simulink model "V1"  (R2025b)
settings: Solver=VariableStepAuto  StartTime=0.0  StopTime=3600*9  RelTol=1e-3
model workspace (MAT data in the model file):
  COP = 3.9
  Delayfan = [30 1]
  P1 = 1.05
  P2 = 1.91
  P3 = 1.91
  P4 = 1.05
  Q_Cond = 4.361
  Q_Evap = 3.471
  T1 = 12
  T2 = 37.72
  T3 = 29.61
  T4 = 7.9
  T_Enviroment_C = 27.5
  T_Room_int_C = 28.6
  T_Tank_int_c = 30
  Wall_h_in = 12
  Wall_h_out = 38
  h1 = 522.3
  h2 = 528.6
  h3 = 253.4
  h4 = 253.4
  m_dot = 0.014
libraries: fl_lib x102, nesl_utility x62, SimscapeFluids_lib x31
(part 1 of 4)
settings Model: Creator=acer  LastModifiedBy=acer

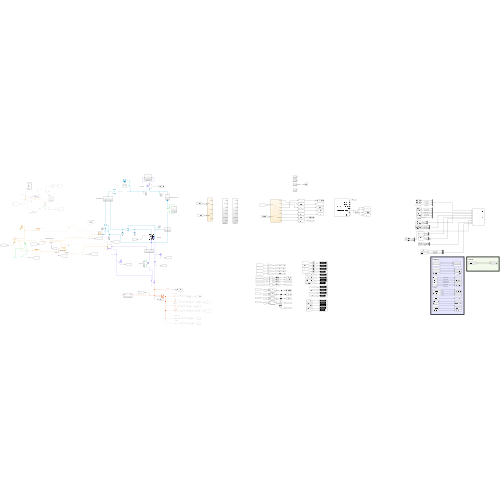
[thumbnail: Simulink's stored preview of the top-level diagram]
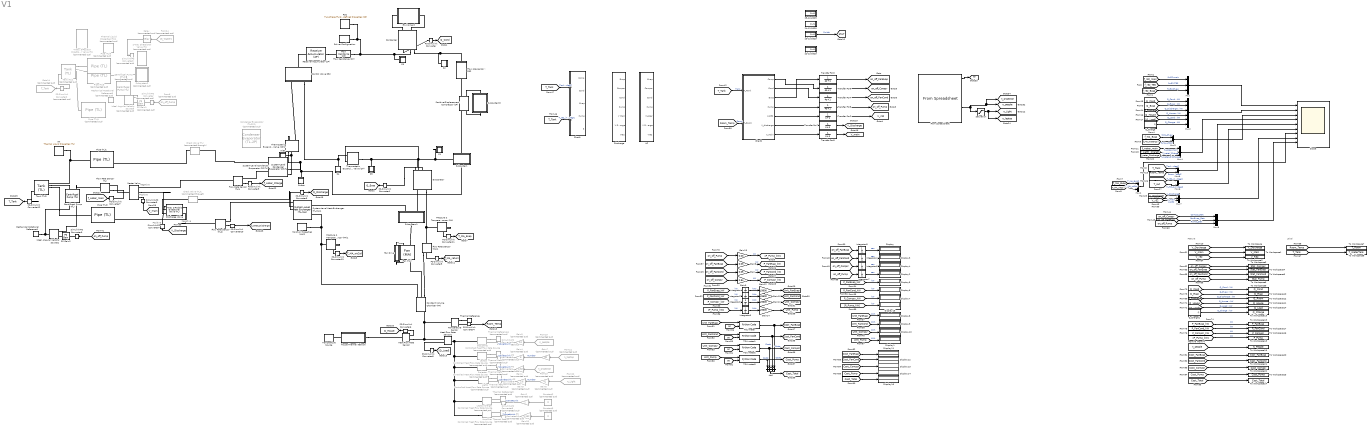
== system V1 ==
  note: Feature
  note: Positive
  note: Negative
  note: Positive
  note: Negative
  note: Label
  2-Way Directional Valve (TL) : SimscapeFluids_lib/Thermal Liquid/Valves & Orifices/Directional Control Valves/2-Way Directional Valve (TL)  Commented=on  valve_spec=fluids.thermal_liquid.valves.directional_control_valves.enum.ValveSpec.Linear  S_max=0.01 m  del_S_max=0.01 m  area_max=0.015 m^2  area_leak=1e-6 m^2  del_S_TLU=[0, .002, .004, .007, .017] m  valve_area_TLU=[1e-09, 2.0352e-07, 4.0736e-05, .00011438, .00034356] m^2  del_S_flow_TLU=[0, .002, .004, .007, .017] m  p_diff_TLU=[.3, .5, .7] MPa  vol_flow_TLU=1e-3 * [1.7e-05, 2e-05, 2.6e-05; .0035, .0045, .0053; .7, .9, 1.06; 1.96, 2.5, 3; 6, 7.7, 9.13] m^3/s  mdot_TLU=[1.7e-05, 2e-05, 2.6e-05; .0035, .0045, .0053; .7, .9, 1.06; 1.96, 2.5, 3; 6, 7.7, 9.13] kg/s  T_ref_in=293.15 K  p_ref_in=0.101325 MPa  Cd=0.9  Re_c=150  smoothing_factor=0.01  pressure_recovery=false  area=0.016 m^2
      settings: InternalSimscapePortConfiguration="{\"Bottom\":[],\"Left\":[{\"id\":\"A\",\"label\":\"A\",\"type\":\"foundation.thermal_liquid.thermal_liquid\"}],\"Right\":[{\"id\":\"S\",\"label\":\"S\",\"type\":\"input\"},{\"id\":\"B\",\"label\":\"B\",\"type\":\"foundation.thermal_liquid.thermal_liquid\"}],\"Top\":[]}"
  22-12-2025 : Subsystem
  23-12-2025 : Subsystem
  24-12-2025 : Subsystem
  25-12-2025 : Subsystem
  4-Way 3-Position Directional Valve (TL) : SimscapeFluids_lib/Thermal Liquid/Valves & Orifices/Directional Control Valves/4-Way 3-Position Directional Valve (TL)  Commented=on  open_orifices_pos=fluids.thermal_liquid.valves.directional_control_valves.enum.OpenOrifices4WayPosNeg.PA  open_orifices_neu=fluids.thermal_liquid.valves.directional_control_valves.enum.OpenOrifices4WayNeu.AT_BT  open_orifices_neg=fluids.thermal_liquid.valves.directional_control_valves.enum.OpenOrifices4WayPosNeg.PA_BT  neutral_assert_action=simscape.enum.assert.action.warn  area_spec=fluids.thermal_liquid.valves.directional_control_valves.enum.area_spec.identical  valve_spec=fluids.thermal_liquid.valves.directional_control_valves.enum.ValveSpec.Linear  del_S_max=0.005 m  area_max=1e-4 m^2  del_S_TLU=[0, .00125, .0025, .00375, .005] m  valve_area_TLU=[1e-10, 1e-05, 4e-05, 6e-05, .0001] m^2  del_S_flow_TLU=[0, .00125, .0025, .00375, .005] m  p_diff_TLU=[-.1, .3, .5, .7] MPa  vol_flow_TLU=[-1e-08, 2.2e-08, 2.8e-08, 3.4e-08; -9e-06, .00015, .0002, .00024; -.00036, .00063, .00081, .00096; -.00054, .00094, .0012, .0014; -.00091, .0016, .002, .0024] m^3/s  mdot_TLU=[-1e-05, 1.7e-05, 2e-05, 2.6e-05; -.009, .0035, .0045, .0053; -.36, .7, .9, 1.06; -.54, 1.96, 2.5, 3; -.91, 6, 7.7, 9.13] kg/s  p_diff_TLU_const=[-.1, .3, .5, .7] MPa  vol_flow_TLU_const=[-.0009, .0016, .002, .0024] m^3/s  mdot_TLU_const=[-.9, 1.6, 2, 2.4] kg/s  area_const=1e-4 m^2  T_ref_in=293.15 K  p_ref_in=0.101325 MPa  area_leak=1e-10 m^2  area=0.01 m^2  Cd=0.64  Re_c=150  smoothing_factor=0.01  pressure_recovery=false  S_max_PA=7.5e-3 m  del_S_max_PA=0.005 m  area_max_PA=1e-4 m^2  del_S_TLU_PA=[0, .00125, .0025, .00375, .005] m  valve_area_TLU_PA=[1e-10, 1e-05, 4e-05, 6e-05, .0001] m^2  del_S_flow_TLU_PA=[0, .00125, .0025, .00375, .005] m  p_diff_TLU_PA=[-.1, .3, .5, .7] MPa  vol_flow_TLU_PA=[-1e-08, 2.2e-08, 2.8e-08, 3.4e-08; -9e-06, .00015, .0002, .00024; -.00036, .00063, .00081, .00096; -.00054, .00094, .0012, .0014; -.00091, .0016, .002, .0024] m^3/s  mdot_TLU_PA=[-1e-05, 1.7e-05, 2e-05, 2.6e-05; -.009, .0035, .0045, .0053; -.36, .7, .9, 1.06; -.54, 1.96, 2.5, 3; -.91, 6, 7.7, 9.13] kg/s  area_const_PA=1e-4 m^2  p_diff_TLU_const_PA=[-.1, .3, .5, .7] MPa  vol_flow_TLU_const_PA=[-.0009, .0016, .002, .0024] m^3/s  mdot_TLU_const_PA=[-.9, 1.6, 2, 2.4] kg/s  S_max_PB=-7.5e-3 m  del_S_max_PB=0.005 m  area_max_PB=1e-4 m^2  del_S_TLU_PB=[0, .00125, .0025, .00375, .005] m  valve_area_TLU_PB=[1e-10, 1e-05, 4e-05, 6e-05, .0001] m^2  del_S_flow_TLU_PB=[0, .00125, .0025, .00375, .005] m  p_diff_TLU_PB=[-.1, .3, .5, .7] MPa  vol_flow_TLU_PB=[-1e-08, 2.2e-08, 2.8e-08, 3.4e-08; -9e-06, .00015, .0002, .00024; -.00036, .00063, .00081, .00096; -.00054, .00094, .0012, .0014; -.00091, .0016, .002, .0024] m^3/s  mdot_TLU_PB=[-1e-05, 1.7e-05, 2e-05, 2.6e-05; -.009, .0035, .0045, .0053; -.36, .7, .9, 1.06; -.54, 1.96, 2.5, 3; -.91, 6, 7.7, 9.13] kg/s  area_const_PB=1e-4 m^2  p_diff_TLU_const_PB=[-.1, .3, .5, .7] MPa  vol_flow_TLU_const_PB=[-.0009, .0016, .002, .0024] m^3/s  mdot_TLU_const_PB=[-.9, 1.6, 2, 2.4] kg/s  S_max_AB=7.5e-3 m  del_S_max_AB=0.005 m  area_max_AB=1e-4 m^2  del_S_TLU_AB=[0, .00125, .0025, .00375, .005] m  valve_area_TLU_AB=[1e-10, 1e-05, 4e-05, 6e-05, .0001] m^2  del_S_flow_TLU_AB=[0, .00125, .0025, .00375, .005] m  p_diff_TLU_AB=[-.1, .3, .5, .7] MPa  vol_flow_TLU_AB=[-1e-08, 2.2e-08, 2.8e-08, 3.4e-08; -9e-06, .00015, .0002, .00024; -.00036, .00063, .00081, .00096; -.00054, .00094, .0012, .0014; -.00091, .0016, .002, .0024] m^3/s  mdot_TLU_AB=[-1e-05, 1.7e-05, 2e-05, 2.6e-05; -.009, .0035, .0045, .0053; -.36, .7, .9, 1.06; -.54, 1.96, 2.5, 3; -.91, 6, 7.7, 9.13] kg/s  area_const_AB=1e-4 m^2  p_diff_TLU_const_AB=[-.1, .3, .5, .7] MPa  vol_flow_TLU_const_AB=[-.0009, .0016, .002, .0024] m^3/s  mdot_TLU_const_AB=[-.9, 1.6, 2, 2.4] kg/s  S_max_AT=-7.5e-3 m  del_S_max_AT=0.005 m  area_max_AT=1e-4 m^2  del_S_TLU_AT=[0, .00125, .0025, .00375, .005] m  valve_area_TLU_AT=[1e-10, 1e-05, 4e-05, 6e-05, .0001] m^2  del_S_flow_TLU_AT=[0, .00125, .0025, .00375, .005] m  p_diff_TLU_AT=[-.1, .3, .5, .7] MPa  vol_flow_TLU_AT=[-1e-08, 2.2e-08, 2.8e-08, 3.4e-08; -9e-06, .00015, .0002, .00024; -.00036, .00063, .00081, .00096; -.00054, .00094, .0012, .0014; -.00091, .0016, .002, .0024] m^3/s  mdot_TLU_AT=[-1e-05, 1.7e-05, 2e-05, 2.6e-05; -.009, .0035, .0045, .0053; -.36, .7, .9, 1.06; -.54, 1.96, 2.5, 3; -.91, 6, 7.7, 9.13] kg/s  area_const_AT=1e-4 m^2  p_diff_TLU_const_AT=[-.1, .3, .5, .7] MPa  vol_flow_TLU_const_AT=[-.0009, .0016, .002, .0024] m^3/s  mdot_TLU_const_AT=[-.9, 1.6, 2, 2.4] kg/s  S_max_BT=7.5e-3 m  del_S_max_BT=0.005 m  area_max_BT=1e-4 m^2  del_S_TLU_BT=[0, .00125, .0025, .00375, .005] m  valve_area_TLU_BT=[1e-10, 1e-05, 4e-05, 6e-05, .0001] m^2  del_S_flow_TLU_BT=[0, .00125, .0025, .00375, .005] m  p_diff_TLU_BT=[-.1, .3, .5, .7] MPa  vol_flow_TLU_BT=[-1e-08, 2.2e-08, 2.8e-08, 3.4e-08; -9e-06, .00015, .0002, .00024; -.00036, .00063, .00081, .00096; -.00054, .00094, .0012, .0014; -.00091, .0016, .002, .0024] m^3/s  mdot_TLU_BT=[-1e-05, 1.7e-05, 2e-05, 2.6e-05; -.009, .0035, .0045, .0053; -.36, .7, .9, 1.06; -.54, 1.96, 2.5, 3; -.91, 6, 7.7, 9.13] kg/s  area_const_BT=1e-4 m^2  p_diff_TLU_const_BT=[-.1, .3, .5, .7] MPa  vol_flow_TLU_const_BT=[-.0009, .0016, .002, .0024] m^3/s  mdot_TLU_const_BT=[-.9, 1.6, 2, 2.4] kg/s  S_max_PT=0 m  del_S_max_PT=0.005 m  area_max_PT=1e-4 m^2  del_S_TLU_PT=[0, .00125, .0025, .00375, .005] m  valve_area_TLU_PT=[1e-10, 1e-05, 4e-05, 6e-05, .0001] m^2  del_S_flow_TLU_PT=[0, .00125, .0025, .00375, .005] m  p_diff_TLU_PT=[-.1, .3, .5, .7] MPa  vol_flow_TLU_PT=[-1e-08, 2.2e-08, 2.8e-08, 3.4e-08; -9e-06, .00015, .0002, .00024; -.00036, .00063, .00081, .00096; -.00054, .00094, .0012, .0014; -.00091, .0016, .002, .0024] m^3/s  mdot_TLU_PT=[-1e-05, 1.7e-05, 2e-05, 2.6e-05; -.009, .0035, .0045, .0053; -.36, .7, .9, 1.06; -.54, 1.96, 2.5, 3; -.91, 6, 7.7, 9.13] kg/s
      settings: InternalSimscapePortConfiguration="{\"Bottom\":[],\"Left\":[{\"id\":\"A\",\"label\":\"A\",\"type\":\"foundation.thermal_liquid.thermal_liquid\"},{\"id\":\"B\",\"label\":\"B\",\"type\":\"foundation.thermal_liquid.thermal_liquid\"}],\"Right\":[{\"id\":\"S\",\"label\":\"S\",\"type\":\"input\"},{\"id\":\"P\",\"label\":\"P\",\"type\":\"foundation.thermal_liquid.thermal_liquid\"},{\"id\":\"T\",\"label\":\"T\",\"type\":\"foundation.thermal_liquid.thermal_liquid\"}],\"Top\":[]}"
  AC : Subsystem
  Add : Sum  Inputs=++++
  Amplifier : fl_lib/Thermal/Thermal Sources/Controlled Heat Flow Rate Source  Commented=on
  Centrifugal Pump (TL) : SimscapeFluids_lib/Thermal Liquid/Pumps & Motors/Centrifugal Pump (TL)  pump_parameterization=fluids.thermal_liquid.pumps_motors.enum.CentrifugalPumpParameterization.Nominal  capacity_ref_nominal=45 lpm  head_ref_nominal=40 m  power_ref_nominal=0.85 kW  head_ref_max=60 m  capacity_ref_max=80 lpm  omega_ref_analytic=1770 rpm  flow_rate_1D_TLU=[16.67, 30, 40, 53.33, 66.67, 83.33] lpm  head_1D_TLU=[50, 47.5, 45, 40, 35, 25] m  power_1D_TLU=[.6, .75, .85, .93, .98, .99] kW  omega_ref_1D=3500 rpm  rho_ref_1D=998.21 kg/m^3  omega_threshold_factor=1e-2  flow_rate_2D_TLU=[16.67, 23.33, 30, 40, 53.33, 60] lpm  omega_2D_TLU=[2450, 2800, 3150, 3500] rpm  head_2D_TLU=[25, 32.7, 42.5, 50; 24, 31.7, 41, 49; 22.7, 30.5, 39, 47.5; 20, 28, 36, 45; 15.7, 24, 32, 40; 12.5, 21, 29.5, 37.5] m  power_2D_TLU=[.28, .38, .5, .6; .31, .41, .55, .68; .33, .44, .6, .75; .36, .48, .65, .83; .38, .53, .72, .93; .39, .55, .75, .97] kW  rho_ref_2D=998.21 kg/m^3  diameter_ratio=1  mech_orientation=fluids.thermal_liquid.pumps_motors.enum.CentrifugalPumpMechOrientation.Positive  area=0.01 m^2  operation_check=simscape.enum.assert.action.none
      settings: InternalSimscapePortConfiguration="{\"Bottom\":[],\"Left\":[{\"id\":\"A\",\"label\":\"A\",\"type\":\"foundation.thermal_liquid.thermal_liquid\"},{\"id\":\"B\",\"label\":\"B\",\"type\":\"foundation.thermal_liquid.thermal_liquid\"}],\"Right\":[{\"id\":\"R\",\"label\":\"R\",\"type\":\"foundation.mechanical.rotational.rotational\"},{\"id\":\"C\",\"label\":\"C\",\"type\":\"foundation.mechanical.rotational.rotational\"}],\"Top\":[]}"
  Centrifugal Pump (TL)2 : SimscapeFluids_lib/Thermal Liquid/Pumps & Motors/Centrifugal Pump (TL)  Commented=on  pump_parameterization=fluids.thermal_liquid.pumps_motors.enum.CentrifugalPumpParameterization.Nominal  capacity_ref_nominal=10 lpm  head_ref_nominal=5 m  power_ref_nominal=0.01 kW  head_ref_max=9 m  capacity_ref_max=11 lpm  omega_ref_analytic=1500 rpm  flow_rate_1D_TLU=[16.67, 30, 40, 53.33, 66.67, 83.33] lpm  head_1D_TLU=[50, 47.5, 45, 40, 35, 25] m  power_1D_TLU=[.6, .75, .85, .93, .98, .99] kW  omega_ref_1D=3500 rpm  rho_ref_1D=998.21 kg/m^3  omega_threshold_factor=1e-2  flow_rate_2D_TLU=[16.67, 23.33, 30, 40, 53.33, 60] lpm  omega_2D_TLU=[2450, 2800, 3150, 3500] rpm  head_2D_TLU=[25, 32.7, 42.5, 50; 24, 31.7, 41, 49; 22.7, 30.5, 39, 47.5; 20, 28, 36, 45; 15.7, 24, 32, 40; 12.5, 21, 29.5, 37.5] m  power_2D_TLU=[.28, .38, .5, .6; .31, .41, .55, .68; .33, .44, .6, .75; .36, .48, .65, .83; .38, .53, .72, .93; .39, .55, .75, .97] kW  rho_ref_2D=998.21 kg/m^3  diameter_ratio=1  mech_orientation=fluids.thermal_liquid.pumps_motors.enum.CentrifugalPumpMechOrientation.Positive  area=7.8e-5 m^2  operation_check=simscape.enum.assert.action.none
      settings: InternalSimscapePortConfiguration="{\"Bottom\":[],\"Left\":[{\"id\":\"A\",\"label\":\"A\",\"type\":\"foundation.thermal_liquid.thermal_liquid\"},{\"id\":\"B\",\"label\":\"B\",\"type\":\"foundation.thermal_liquid.thermal_liquid\"}],\"Right\":[{\"id\":\"R\",\"label\":\"R\",\"type\":\"foundation.mechanical.rotational.rotational\"},{\"id\":\"C\",\"label\":\"C\",\"type\":\"foundation.mechanical.rotational.rotational\"}],\"Top\":[]}"
  Chart1 : Stateflow chart  TreatAsAtomicUnit=on
  Chart2 : Stateflow chart  TreatAsAtomicUnit=on
  Check Valve (TL) : SimscapeFluids_lib/Thermal Liquid/Valves & Orifices/Directional Control Valves/Check Valve (TL)  Commented=through  opening_spec=fluids.thermal_liquid.valves.enum.PressureOpeningSpec.Linear  pressure_spec=fluids.thermal_liquid.valves.enum.PressureControlSpec.PressureDifferential  p_crack_gauge=0.1 MPa  p_crack_differential=0.01 MPa  press_max_gauge=0.2 MPa  press_max_differential=0.02 MPa  area_max=1e-4 m^2  area_leak=1e-10 m^2  p_diff_TLU=[0.01 : 0.01 : 0.1] MPa  valve_area_TLU=[1e-10, 1e-05, 2e-05, 3e-05, 4e-05, 5e-05, 6e-05, 7.5e-05, 8.5e-05, .0001] m^2  vol_flow_TLU=[.000358, .045, .11, .191, .284, .39, .505, .63, .764, .905] .* 1e-3 m^3/s  area=0.01 m^2  Cd=0.64  Re_c=150  smoothing_factor=0.01  pressure_recovery=false  opening_dynamics=false  tau=0.1 s
      settings: InternalSimscapePortConfiguration="{\"Bottom\":[],\"Left\":[{\"id\":\"A\",\"label\":\"A\",\"type\":\"foundation.thermal_liquid.thermal_liquid\"}],\"Right\":[{\"id\":\"B\",\"label\":\"B\",\"type\":\"foundation.thermal_liquid.thermal_liquid\"}],\"Top\":[]}"
  Check Valve (TL)1 : SimscapeFluids_lib/Thermal Liquid/Valves & Orifices/Directional Control Valves/Check Valve (TL)  Commented=through  opening_spec=fluids.thermal_liquid.valves.enum.PressureOpeningSpec.Linear  pressure_spec=fluids.thermal_liquid.valves.enum.PressureControlSpec.PressureDifferential  p_crack_gauge=0.1 MPa  p_crack_differential=0.01 MPa  press_max_gauge=0.2 MPa  press_max_differential=0.02 MPa  area_max=1e-4 m^2  area_leak=1e-10 m^2  p_diff_TLU=[0.01 : 0.01 : 0.1] MPa  valve_area_TLU=[1e-10, 1e-05, 2e-05, 3e-05, 4e-05, 5e-05, 6e-05, 7.5e-05, 8.5e-05, .0001] m^2  vol_flow_TLU=[.000358, .045, .11, .191, .284, .39, .505, .63, .764, .905] .* 1e-3 m^3/s  area=0.01 m^2  Cd=0.64  Re_c=150  smoothing_factor=0.01  pressure_recovery=false  opening_dynamics=false  tau=0.1 s
      settings: InternalSimscapePortConfiguration="{\"Bottom\":[],\"Left\":[{\"id\":\"A\",\"label\":\"A\",\"type\":\"foundation.thermal_liquid.thermal_liquid\"}],\"Right\":[{\"id\":\"B\",\"label\":\"B\",\"type\":\"foundation.thermal_liquid.thermal_liquid\"}],\"Top\":[]}"
  Condenser : SimscapeFluids_lib/Heat Exchangers/Two-Phase Fluid - Moist Air/System-Level Condenser Evaporator (2P-MA)  flow_arrangement=fluids.heat_exchangers.enum.SystemLevelFlowArrangement2PMA.Counter  wall_thermal_mass=false  mass_wall=1 kg  cp_wall=490 J/(K*kg)  nominal_init_wall=true  T_wall_init=293.15 K  area_A1=0.01 m^2  area_B1=0.01 m^2  area_A2=0.01 m^2  area_B2=0.01 m^2  operating_condition_2P=fluids.heat_exchangers.enum.SystemLevelOperatingCondition2PMA.Condenser  mdot_nominal_2P=m_dot kg/s  delta_p_nominal_2P=0.045 MPa  pressure_spec_cond_2P=fluids.heat_exchangers.enum.SystemLevelPressureSpecCondenser2P.InletPressure  pressure_spec_evap_2P=fluids.heat_exchangers.enum.SystemLevelPressureSpecEvaporator2P.InletPressure  p_in_nominal_2P=P2 MPa  T_cond_nominal_2P=313.15 K  T_evap_nominal_2P=243.15 K  inlet_spec_2P=fluids.heat_exchangers.enum.SystemLevelInletSpec2P.Enthalpy  T_in_nominal_2P=333.15 K  h_in_nominal_2P=h2 kJ/kg  x_in_nominal_2P=1  capacity_spec_2P=fluids.heat_exchangers.enum.SystemLevelCapacitySpec.HeatTransfer  Q_nominal=m_dot*(h2-h3) kW  outlet_spec_cond_2P=fluids.heat_exchangers.enum.SystemLevelOutletSpecCondenser2P.Enthalpy  outlet_spec_evap_2P=fluids.heat_exchangers.enum.SystemLevelOutletSpecEvaporator2P.Enthalpy  delta_T_sub_nominal_2P=5 deltaK  delta_T_sup_nominal_2P=5 deltaK  h_out_nominal_2P=250 kJ/kg  x_out_nominal_2P=0  volume_2P=0.001 m^3  nominal_init_2P=true  energy_spec_2P=foundation.enum.energy_spec.enthalpy  p_init_2P=0.101325 MPa  T_init_2P=293.15 K  x_init_2P=0.5  alpha_init_2P=0.5  h_init_2P=1500 kJ/kg  u_init_2P=1500 kJ/kg  mdot_nominal_MA=5 kg/s  delta_p_nominal_MA=0.001 MPa  p_in_nominal_MA=0.101325 MPa  T_in_nominal_MA=T_Enviroment_C+273.15 K  inlet_humidity_spec_MA=foundation.enum.HumiditySpec.RelativeHumidity  RH_in_nominal_MA=0.5  x_w_in_nominal_MA=0.01  y_w_in_nominal_MA=0.01  HR_in_nominal_MA=0.01  Tw_in_nominal_MA=287 K  inlet_trace_gas_spec_MA=foundation.enum.trace_gas_spec.mass_fraction  x_g_in_nominal_MA=0.001  y_g_in_nominal_MA=0.001  volume_MA=0.1 m^3  nominal_init_MA=true  p_init_MA=0.101325 MPa  T_init_MA=293.15 K  humidity_spec_MA=foundation.enum.HumiditySpec.RelativeHumidity  RH_init_MA=0.5  x_w_init_MA=0.01  y_w_init_MA=0.01  HR_init_MA=0.01  Tw_init_MA=287 K  trace_gas_spec_MA=foundation.enum.trace_gas_spec.mass_fraction  x_g_init_MA=0.001  y_g_init_MA=0.001  r_d_init_MA=0  RH_ws_MA=1  time_constant_cond_MA=1e-3 s  time_constant_evap_MA=1e-3 s  fraction_entrained_MA=1  a_liq_2P=0.023  a_mix_2P=0.005  a_vap_2P=0.023  b_2P=0.8  c_2P=0.33  a_MA=0.023  b_MA=0.8  c_MA=0.33
      settings: InternalSimscapePortConfiguration="{\"Bottom\":[],\"Left\":[{\"id\":\"A1\",\"label\":\"A1\",\"type\":\"foundation.two_phase_fluid.two_phase_fluid\"},{\"id\":\"B1\",\"label\":\"B1\",\"type\":\"foundation.two_phase_fluid.two_phase_fluid\"}],\"Right\":[{\"id\":\"A2\",\"label\":\"A2\",\"type\":\"foundation.moist_air.moist_air\"},{\"id\":\"B2\",\"label\":\"B2\",\"type\":\"foundation.moist_air.moist_air\"}],\"Top\":[{\"id\":\"Q1\",\"label\":\"Q1\",\"type\":\"output\"},{\"id\":\"Q2\",\"label\":\"Q2\",\"type\":\"output\"},{\"id\":\"W\",\"label\":\"W\",\"type\":\"output\"}]}"
  Condenser Evaporator (TL-2P)1 : SimscapeFluids_lib/Heat Exchangers/Two-Phase Fluid - Thermal Liquid/Condenser Evaporator (TL-2P)  Commented=on  flow_arrangement=fluids.heat_exchangers.enum.FlowArrangementTL2P.Counter  cross_flow_arrangement=fluids.heat_exchangers.enum.CrossFlowArrangementTL2P.UnmixedUnmixed  R_wall=0.1 K/kW  wall_thermal_mass=true  mass_wall=4 kg  cp_wall=600 J/(K*kg)  area_A1=0.01 m^2  area_B1=0.01 m^2  area_A2=0.01 m^2  area_B2=0.01 m^2  flow_geometry_TL=fluids.heat_exchangers.enum.FlowGeometryTL.InsideTubes  tube_num_TL=30  tube_length_TL=2 m  tube_cross_section_TL=fluids.heat_exchangers.enum.TubeCrossSection.Circular  tube_diameter_TL=0.01 m  tube_width_TL=0.05 m  tube_height_TL=0.05 m  tube_inner_diameter_TL=0.05 m  tube_outer_diameter_TL=0.1 m  tube_flow_area_TL=0.002 m^2  tube_wetted_perimeter_TL=0.15 m  tube_heat_perimeter_TL=0.15 m  tube_pressure_loss_spec_TL=fluids.heat_exchangers.enum.TubePressureLossSpec.Haaland  tube_loss_coeff_TL=10  tube_local_pressure_loss_spec_TL=fluids.heat_exchangers.enum.LocalLossSpec.AggregateLength  tube_length_add_TL=0.1 m  tube_local_loss_coefficient_TL=0.1  tube_roughness_pressure_TL=15e-6 m  tube_Re_lam_pressure_TL=2000  tube_Re_tur_pressure_TL=4000  tube_shape_factor_generic_TL=64  tube_heat_coeff_spec_TL=fluids.heat_exchangers.enum.TubeHeatCoeffSpec.Gneilinski  tube_colburn_coeff_TL=[.023, .8, .33]  tube_roughness_heat_TL=15e-6 m  tube_Re_lam_heat_TL=2000  tube_Re_tur_heat_TL=4000  tube_Nu_lam_generic_TL=3.66  bank_arrangement_TL=fluids.heat_exchangers.enum.BankArrangement.Inline  bank_num_rows_TL=5  bank_tubes_per_row_TL=5  bank_width_TL=1 m  bank_tube_diameter_TL=0.05 m  bank_longitudinal_pitch_TL=0.15 m  bank_transverse_pitch_TL=0.15 m  bank_pressure_loss_spec_TL=fluids.heat_exchangers.enum.BankPressureLossSpec.Martin  bank_euler_TL=10  bank_heat_coeff_spec_TL=fluids.heat_exchangers.enum.BankHeatCoeffSpec.Martin  bank_colburn_coeff_TL=[.27, .63, .36]  generic_flow_area_TL=0.01 m^2  generic_heat_area_TL=2 m^2  generic_volume_TL=0.05 m^3  generic_loss_coeff_TL=10  generic_colburn_coeff_TL=[.023, .8, .33]  fouling_factor_TL=0.001 K*m^2/kW  fin_area_TL=0 m^2  fin_efficiency_TL=0.5  p_init_TL=0.101325 MPa  T_init_TL=30 degC  tube_num_2P=30  tube_length_2P=2 m  tube_cross_section_2P=fluids.heat_exchangers.enum.TubeCrossSection.Circular  tube_diameter_2P=0.01 m  tube_width_2P=0.05 m  tube_height_2P=0.05 m  tube_inner_diameter_2P=0.05 m  tube_outer_diameter_2P=0.1 m  tube_flow_area_2P=0.002 m^2  tube_wetted_perimeter_2P=0.15 m  tube_heat_perimeter_2P=0.15 m  tube_pressure_loss_spec_2P=fluids.heat_exchangers.enum.TubePressureLossSpec2P.Haaland  tube_loss_coeff_2P=10  tube_local_pressure_loss_spec_2P=fluids.heat_exchangers.enum.LocalLossSpec.AggregateLength  tube_length_add_2P=0.1 m  tube_local_loss_coefficient_2P=0.1  tube_roughness_pressure_2P=15e-6 m  tube_Re_lam_pressure_2P=2000  tube_Re_tur_pressure_2P=4000  tube_shape_factor_generic_2P=64  tube_heat_coeff_spec_2P=fluids.heat_exchangers.enum.TubeHeatCoeffSpec2P.GneilinskiCavalliniZecchin  tube_colburn_coeff_liq_2P=[.023, .8, .33]  tube_colburn_coeff_mix_2P=[.05, .8, .33]  tube_colburn_coeff_vap_2P=[.023, .8, .33]  tube_roughness_heat_2P=15e-6 m  tube_Re_lam_heat_2P=2000  tube_Re_tur_heat_2P=4000  tube_Nu_lam_generic_2P=3.66  fouling_factor_2P=0.1 K*m^2/kW  fin_area_2P=0 m^2  fin_efficiency_2P=0.5  energy_spec_2P=foundation.enum.energy_spec.temperature  p_init_2P=0.619 MPa  T_init_2P=6.8 degC  x_init_2P=0.5  alpha_init_2P=0.5  h_init_2P=1500 kJ/kg  u_init_2P=1500 kJ/kg
      settings: InternalSimscapePortConfiguration="{\"Bottom\":[],\"Left\":[{\"id\":\"A1\",\"label\":\"A1\",\"type\":\"foundation.thermal_liquid.thermal_liquid\"},{\"id\":\"B1\",\"label\":\"B1\",\"type\":\"foundation.thermal_liquid.thermal_liquid\"}],\"Right\":[{\"id\":\"A2\",\"label\":\"A2\",\"type\":\"foundation.two_phase_fluid.two_phase_fluid\"},{\"id\":\"B2\",\"label\":\"B2\",\"type\":\"foundation.two_phase_fluid.two_phase_fluid\"}],\"Top\":[{\"id\":\"Z\",\"label\":\"Z\",\"type\":\"output\"}]}"
  Constant Volume Chamber (MA) : fl_lib/Moist Air/Elements/Constant Volume Chamber (MA)  volume=92.924*1.5 m^3  num_ports=foundation.enum.num_ports.three  area_A=0.01 m^2  area_B=0.01 m^2  area_C=0.01 m^2  area_D=0.01 m^2  RH_ws=1  time_constant_cond=1e-3 s  time_constant_evap=1e-3 s  fraction_entrained=1  moisture_trace_gas_source=foundation.enum.moisture_trace_gas_source.none  moisture_source_spec=foundation.enum.MoistureSourceSpec.WaterVapor  vapor_from_liquid=false  moisture_mass_flow=0 kg/s  moisture_temperature_spec=foundation.enum.temperature_spec.atmospheric  moisture_temperature=293.15 K  trace_gas_mass_flow=0 kg/s  trace_gas_temperature_spec=foundation.enum.temperature_spec.atmospheric  trace_gas_temperature=293.15 K  p_init=0.101325 MPa  p_init_priority=foundation.enum.Priority.High  T_init=273.15+T_Room_int_C K  T_init_priority=foundation.enum.Priority.High  humidity_spec=foundation.enum.HumiditySpec.RelativeHumidity  RH_init=0.5  RH_init_priority=foundation.enum.Priority.High  x_w_init=0.01  x_w_init_priority=foundation.enum.Priority.High  y_w_init=0.01  y_w_init_priority=foundation.enum.Priority.High  HR_init=0.01  HR_init_priority=foundation.enum.Priority.High  Tw_init=287 K  Tw_init_priority=foundation.enum.Priority.High  trace_gas_spec=foundation.enum.trace_gas_spec.mass_fraction  x_g_init=0.001  x_g_init_priority=foundation.enum.Priority.High  y_g_init=0.001  y_g_init_priority=foundation.enum.Priority.High  r_d_init=0  r_d_init_priority=foundation.enum.Priority.High
      settings: InternalSimscapePortConfiguration="{\"Bottom\":[],\"Left\":[{\"id\":\"A\",\"label\":\"A\",\"type\":\"foundation.moist_air.moist_air\"},{\"id\":\"B\",\"label\":\"B\",\"type\":\"foundation.moist_air.moist_air\"},{\"id\":\"C\",\"label\":\"C\",\"type\":\"foundation.moist_air.moist_air\"}],\"Right\":[{\"id\":\"W\",\"label\":\"W\",\"type\":\"output\"},{\"id\":\"F\",\"label\":\"F\",\"type\":\"output\"},{\"id\":\"H\",\"label\":\"H\",\"type\":\"foundation.thermal.thermal\"}],\"Top\":[]}"
  Constant2 : Constant  Commented=on  Value=0
  Constant3 : Constant  Commented=on  Value=0
  Control Valve R32 : Subsystem
  Discharge : Subsystem
  Discharge Valve : SimscapeFluids_lib/Thermal Liquid/Valves & Orifices/Directional Control Valves/4-Way 2-Position Directional Valve (TL)  open_orifices_pos=fluids.thermal_liquid.valves.directional_control_valves.enum.OpenOrifices4Way2Position.PA_BT  open_orifices_neg=fluids.thermal_liquid.valves.directional_control_valves.enum.OpenOrifices4Way2Position.PB_AT  area_spec=fluids.thermal_liquid.valves.directional_control_valves.enum.area_spec.identical  valve_spec=fluids.thermal_liquid.valves.directional_control_valves.enum.ValveSpec.Linear  del_S_max=0.01 m  area_max=0.012 m^2  del_S_TLU=[0, .00125, .0025, .00375, .005] m  valve_area_TLU=[1e-10, 1e-05, 4e-05, 6e-05, .0001] m^2  del_S_flow_TLU=[0, .00125, .0025, .00375, .005] m  p_diff_TLU=[-.1, .3, .5, .7] MPa  vol_flow_TLU=[-1e-08, 2.2e-08, 2.8e-08, 3.4e-08; -9e-06, .00015, .0002, .00024; -.00036, .00063, .00081, .00096; -.00054, .00094, .0012, .0014; -.00091, .0016, .002, .0024] m^3/s  mdot_TLU=[-1e-05, 1.7e-05, 2e-05, 2.6e-05; -.009, .0035, .0045, .0053; -.36, .7, .9, 1.06; -.54, 1.96, 2.5, 3; -.91, 6, 7.7, 9.13] kg/s  p_diff_TLU_const=[-.1, .3, .5, .7] MPa  vol_flow_TLU_const=[-.0009, .0016, .002, .0024] m^3/s  mdot_TLU_const=[-.9, 1.6, 2, 2.4] kg/s  area_const=1e-4 m^2  T_ref_in=293.15 K  p_ref_in=0.101325 MPa  area_leak=1e-10 m^2  area=0.015 m^2  Cd=0.64  Re_c=150  smoothing_factor=0.01  pressure_recovery=false  S_max_PA=0.01 m  del_S_max_PA=0.005 m  area_max_PA=1e-4 m^2  del_S_TLU_PA=[0, .00125, .0025, .00375, .005] m  valve_area_TLU_PA=[1e-10, 1e-05, 4e-05, 6e-05, .0001] m^2  del_S_flow_TLU_PA=[0, .00125, .0025, .00375, .005] m  p_diff_TLU_PA=[-.1, .3, .5, .7] MPa  vol_flow_TLU_PA=[-1e-08, 2.2e-08, 2.8e-08, 3.4e-08; -9e-06, .00015, .0002, .00024; -.00036, .00063, .00081, .00096; -.00054, .00094, .0012, .0014; -.00091, .0016, .002, .0024] m^3/s  mdot_TLU_PA=[-1e-05, 1.7e-05, 2e-05, 2.6e-05; -.009, .0035, .0045, .0053; -.36, .7, .9, 1.06; -.54, 1.96, 2.5, 3; -.91, 6, 7.7, 9.13] kg/s  area_const_PA=1e-4 m^2  p_diff_TLU_const_PA=[-.1, .3, .5, .7] MPa  vol_flow_TLU_const_PA=[-.0009, .0016, .002, .0024] m^3/s  mdot_TLU_const_PA=[-.9, 1.6, 2, 2.4] kg/s  S_max_PB=0.01 m  del_S_max_PB=0.005 m  area_max_PB=1e-4 m^2  del_S_TLU_PB=[0, .00125, .0025, .00375, .005] m  valve_area_TLU_PB=[1e-10, 1e-05, 4e-05, 6e-05, .0001] m^2  del_S_flow_TLU_PB=[0, .00125, .0025, .00375, .005] m  p_diff_TLU_PB=[-.1, .3, .5, .7] MPa  vol_flow_TLU_PB=[-1e-08, 2.2e-08, 2.8e-08, 3.4e-08; -9e-06, .00015, .0002, .00024; -.00036, .00063, .00081, .00096; -.00054, .00094, .0012, .0014; -.00091, .0016, .002, .0024] m^3/s  mdot_TLU_PB=[-1e-05, 1.7e-05, 2e-05, 2.6e-05; -.009, .0035, .0045, .0053; -.36, .7, .9, 1.06; -.54, 1.96, 2.5, 3; -.91, 6, 7.7, 9.13] kg/s  area_const_PB=1e-4 m^2  p_diff_TLU_const_PB=[-.1, .3, .5, .7] MPa  vol_flow_TLU_const_PB=[-.0009, .0016, .002, .0024] m^3/s  mdot_TLU_const_PB=[-.9, 1.6, 2, 2.4] kg/s  S_max_AT=0.01 m  del_S_max_AT=0.005 m  area_max_AT=1e-4 m^2  del_S_TLU_AT=[0, .00125, .0025, .00375, .005] m  valve_area_TLU_AT=[1e-10, 1e-05, 4e-05, 6e-05, .0001] m^2  del_S_flow_TLU_AT=[0, .00125, .0025, .00375, .005] m  p_diff_TLU_AT=[-.1, .3, .5, .7] MPa  vol_flow_TLU_AT=[-1e-08, 2.2e-08, 2.8e-08, 3.4e-08; -9e-06, .00015, .0002, .00024; -.00036, .00063, .00081, .00096; -.00054, .00094, .0012, .0014; -.00091, .0016, .002, .0024] m^3/s  mdot_TLU_AT=[-1e-05, 1.7e-05, 2e-05, 2.6e-05; -.009, .0035, .0045, .0053; -.36, .7, .9, 1.06; -.54, 1.96, 2.5, 3; -.91, 6, 7.7, 9.13] kg/s  area_const_AT=1e-4 m^2  p_diff_TLU_const_AT=[-.1, .3, .5, .7] MPa  vol_flow_TLU_const_AT=[-.0009, .0016, .002, .0024] m^3/s  mdot_TLU_const_AT=[-.9, 1.6, 2, 2.4] kg/s  S_max_BT=0.01 m  del_S_max_BT=0.005 m  area_max_BT=1e-4 m^2  del_S_TLU_BT=[0, .00125, .0025, .00375, .005] m  valve_area_TLU_BT=[1e-10, 1e-05, 4e-05, 6e-05, .0001] m^2  del_S_flow_TLU_BT=[0, .00125, .0025, .00375, .005] m  p_diff_TLU_BT=[-.1, .3, .5, .7] MPa  vol_flow_TLU_BT=[-1e-08, 2.2e-08, 2.8e-08, 3.4e-08; -9e-06, .00015, .0002, .00024; -.00036, .00063, .00081, .00096; -.00054, .00094, .0012, .0014; -.00091, .0016, .002, .0024] m^3/s  mdot_TLU_BT=[-1e-05, 1.7e-05, 2e-05, 2.6e-05; -.009, .0035, .0045, .0053; -.36, .7, .9, 1.06; -.54, 1.96, 2.5, 3; -.91, 6, 7.7, 9.13] kg/s  area_const_BT=1e-4 m^2  p_diff_TLU_const_BT=[-.1, .3, .5, .7] MPa  vol_flow_TLU_const_BT=[-.0009, .0016, .002, .0024] m^3/s  mdot_TLU_const_BT=[-.9, 1.6, 2, 2.4] kg/s
      settings: InternalSimscapePortConfiguration="{\"Bottom\":[{\"id\":\"P\",\"label\":\"P\",\"type\":\"foundation.thermal_liquid.thermal_liquid\"},{\"id\":\"T\",\"label\":\"T\",\"type\":\"foundation.thermal_liquid.thermal_liquid\"}],\"Left\":[{\"id\":\"S\",\"label\":\"S\",\"type\":\"input\"}],\"Right\":[],\"Top\":[{\"id\":\"A\",\"label\":\"A\",\"type\":\"foundation.thermal_liquid.thermal_liquid\"},{\"id\":\"B\",\"label\":\"B\",\"type\":\"foundation.thermal_liquid.thermal_liquid\"}]}"
  Display{,1..16} (17 alike) : Display
  Enviroment : Subsystem
  Evaporator : SimscapeFluids_lib/Heat Exchangers/Two-Phase Fluid - Moist Air/System-Level Condenser Evaporator (2P-MA)  flow_arrangement=fluids.heat_exchangers.enum.SystemLevelFlowArrangement2PMA.Counter  wall_thermal_mass=false  mass_wall=1 kg  cp_wall=490 J/(K*kg)  nominal_init_wall=true  T_wall_init=293.15 K  area_A1=0.01 m^2  area_B1=0.01 m^2  area_A2=0.01 m^2  area_B2=0.01 m^2  operating_condition_2P=fluids.heat_exchangers.enum.SystemLevelOperatingCondition2PMA.Evaporator  mdot_nominal_2P=m_dot kg/s  delta_p_nominal_2P=0.03 MPa  pressure_spec_cond_2P=fluids.heat_exchangers.enum.SystemLevelPressureSpecCondenser2P.InletPressure  pressure_spec_evap_2P=fluids.heat_exchangers.enum.SystemLevelPressureSpecEvaporator2P.InletPressure  p_in_nominal_2P=P4 MPa  T_cond_nominal_2P=313.15 K  T_evap_nominal_2P=243.15 K  inlet_spec_2P=fluids.heat_exchangers.enum.SystemLevelInletSpec2P.Enthalpy  T_in_nominal_2P=333.15 K  h_in_nominal_2P=h4 kJ/kg  x_in_nominal_2P=1  capacity_spec_2P=fluids.heat_exchangers.enum.SystemLevelCapacitySpec.HeatTransfer  Q_nominal=m_dot*(h1-h4) kW  outlet_spec_cond_2P=fluids.heat_exchangers.enum.SystemLevelOutletSpecCondenser2P.Enthalpy  outlet_spec_evap_2P=fluids.heat_exchangers.enum.SystemLevelOutletSpecEvaporator2P.Enthalpy  delta_T_sub_nominal_2P=5 deltaK  delta_T_sup_nominal_2P=5 deltaK  h_out_nominal_2P=250 kJ/kg  x_out_nominal_2P=0  volume_2P=0.001 m^3  nominal_init_2P=true  energy_spec_2P=foundation.enum.energy_spec.enthalpy  p_init_2P=0.101325 MPa  T_init_2P=293.15 K  x_init_2P=0.5  alpha_init_2P=0.5  h_init_2P=1500 kJ/kg  u_init_2P=1500 kJ/kg  mdot_nominal_MA=0.44 kg/s  delta_p_nominal_MA=0.001 MPa  p_in_nominal_MA=0.101325 MPa  T_in_nominal_MA=292.65 K  inlet_humidity_spec_MA=foundation.enum.HumiditySpec.RelativeHumidity  RH_in_nominal_MA=0.5  x_w_in_nominal_MA=0.01  y_w_in_nominal_MA=0.01  HR_in_nominal_MA=0.01  Tw_in_nominal_MA=287 K  inlet_trace_gas_spec_MA=foundation.enum.trace_gas_spec.mass_fraction  x_g_in_nominal_MA=0.001  y_g_in_nominal_MA=0.001  volume_MA=0.1 m^3  nominal_init_MA=true  p_init_MA=0.101325 MPa  T_init_MA=293.15 K  humidity_spec_MA=foundation.enum.HumiditySpec.RelativeHumidity  RH_init_MA=0.5  x_w_init_MA=0.01  y_w_init_MA=0.01  HR_init_MA=0.01  Tw_init_MA=287 K  trace_gas_spec_MA=foundation.enum.trace_gas_spec.mass_fraction  x_g_init_MA=0.001  y_g_init_MA=0.001  r_d_init_MA=0  RH_ws_MA=1  time_constant_cond_MA=1e-3 s  time_constant_evap_MA=1e-3 s  fraction_entrained_MA=1  a_liq_2P=0.023  a_mix_2P=0.005  a_vap_2P=0.023  b_2P=0.8  c_2P=0.33  a_MA=0.023  b_MA=0.8  c_MA=0.33
      settings: InternalSimscapePortConfiguration="{\"Bottom\":[],\"Left\":[{\"id\":\"A1\",\"label\":\"A1\",\"type\":\"foundation.two_phase_fluid.two_phase_fluid\"},{\"id\":\"B1\",\"label\":\"B1\",\"type\":\"foundation.two_phase_fluid.two_phase_fluid\"}],\"Right\":[{\"id\":\"A2\",\"label\":\"A2\",\"type\":\"foundation.moist_air.moist_air\"},{\"id\":\"B2\",\"label\":\"B2\",\"type\":\"foundation.moist_air.moist_air\"}],\"Top\":[{\"id\":\"Q1\",\"label\":\"Q1\",\"type\":\"output\"},{\"id\":\"Q2\",\"label\":\"Q2\",\"type\":\"output\"},{\"id\":\"W\",\"label\":\"W\",\"type\":\"output\"}]}"
  Fan (MA) : SimscapeFluids_lib/Moist Air/Turbomachinery/Fan (MA)  fan_parameterization=fluids.moist_air.turbomachinery.enum.FanParameterization.Nominal  mechanical_power_spec=fluids.moist_air.turbomachinery.enum.FanMechanicalPowerSpec.Efficiency  flow_rate_nominal=0.6+0.14 m^3/s  pressure_nominal=5400 Pa  eta_nominal=0.40  power_nominal=1620 W  pressure_max=6400 Pa  flow_rate_max=0.602+0.14 m^3/s  omega_ref_nominal=1200 rpm  flow_rate_1D_TLU=[.0278, .0556, .0833, .111, .139, .167] m^3/s  pressure_1D_TLU=[6410, 6375, 6018, 5366, 4501, 3609] Pa  eta_1D_TLU=[.257, .394, .453, .47, .459, .415]  power_1D_TLU=[693, 900, 1107, 1267, 1363, 1452] W  omega_ref_1D=3000 rpm  rho_ref_1D=1.2 kg/m^3  omega_threshold_factor=1e-2  omega_dp_TLU=[2400; 3000; 3600] rpm  flow_rate_dp_TLU=[.0278, .0556, .0833, .111, .139, .167] m^3/s  pressure_dp_TLU=[4111, 4010, 3551, 2881, 2167, 1453; 6410, 6375, 6018, 5366, 4501, 3609; 9217, 9285, 9022, 8428, 7552, 6482] Pa  eta_dp_TLU=[.3, .434, .468, .459, .4, .3; .257, .394, .453, .47, .459, .415; .225, .359, .434, .461, .47, .459]  power_dp_TLU=[381, 514, 632, 697, 753, 809; 693, 900, 1107, 1267, 1363, 1452; 1139, 1438, 1732, 2029, 2233, 2358] W  rho_ref_dp=1.2 kg/m^3  omega_q_TLU=[2990; 3450; 3867] rpm  pressure_q_TLU=[31, 62, 93, 124] Pa  flow_rate_q_TLU=[.802, .759, .703, .611; .936, .902, .862, .81; 1.056, 1.027, .994, .956] m^3/s  eta_q_TLU=[.088, .162, .22, .261; .068, .128, .18, .222; .055, .105, .148, .188]  power_q_TLU=[283, 290, 297, 290; 427, 437, 445, 452; 595, 606, 625, 631] W  rho_ref_q=1.2 kg/m^3  diameter_ratio=1  mech_orientation=fluids.moist_air.turbomachinery.enum.FanMechanicalOrientation.Positive  area_A=0.01 m^2  area_B=0.01 m^2
      settings: InternalSimscapePortConfiguration="{\"Bottom\":[],\"Left\":[{\"id\":\"A\",\"label\":\"A\",\"type\":\"foundation.moist_air.moist_air\"},{\"id\":\"C\",\"label\":\"C\",\"type\":\"foundation.mechanical.rotational.rotational\"}],\"Right\":[{\"id\":\"B\",\"label\":\"B\",\"type\":\"foundation.moist_air.moist_air\"},{\"id\":\"R\",\"label\":\"R\",\"type\":\"foundation.mechanical.rotational.rotational\"}],\"Top\":[]}"
  Fan Drive : Subsystem
  Flow Rate Sensor (MA)1 : fl_lib/Moist Air/Sensors/Flow Rate Sensor (MA)  mass_flow_measure=true  volumetric_flow_measure=false  volumetric_flow_conditions=foundation.enum.volumetric_flow_conditions.actual  p_std=0.101325 MPa  T_std=20 degC  RH_std=0.65  energy_flow_measure=true  vapor_flow_measure=false  gas_flow_measure=false  droplets_flow_measure=false
      settings: InternalSimscapePortConfiguration="{\"Bottom\":[{\"id\":\"PHI\",\"label\":\"φ\",\"type\":\"output\"}],\"Left\":[{\"id\":\"A\",\"label\":\"A\",\"type\":\"foundation.moist_air.moist_air\"}],\"Right\":[{\"id\":\"B\",\"label\":\"B\",\"type\":\"foundation.moist_air.moist_air\"},{\"id\":\"M\",\"label\":\"M\",\"type\":\"output\"}],\"Top\":[]}"
  Flow Rate Sensor (TL) : fl_lib/Thermal Liquid/Sensors/Flow Rate Sensor (TL)  mass_flow_measure=true  volumetric_flow_measure=false  energy_flow_measure=false
      settings: InternalSimscapePortConfiguration="{\"Bottom\":[],\"Left\":[{\"id\":\"A\",\"label\":\"A\",\"type\":\"foundation.thermal_liquid.thermal_liquid\"}],\"Right\":[{\"id\":\"B\",\"label\":\"B\",\"type\":\"foundation.thermal_liquid.thermal_liquid\"},{\"id\":\"M\",\"label\":\"M\",\"type\":\"output\"}],\"Top\":[]}"
  Flow Rate Sensor (TL)1 : fl_lib/Thermal Liquid/Sensors/Flow Rate Sensor (TL)  mass_flow_measure=true  volumetric_flow_measure=false  energy_flow_measure=false
      settings: InternalSimscapePortConfiguration="{\"Bottom\":[],\"Left\":[{\"id\":\"A\",\"label\":\"A\",\"type\":\"foundation.thermal_liquid.thermal_liquid\"}],\"Right\":[{\"id\":\"B\",\"label\":\"B\",\"type\":\"foundation.thermal_liquid.thermal_liquid\"},{\"id\":\"M\",\"label\":\"M\",\"type\":\"output\"}],\"Top\":[]}"
  Flow Rate Sensor (TL)2 : fl_lib/Thermal Liquid/Sensors/Flow Rate Sensor (TL)  mass_flow_measure=true  volumetric_flow_measure=false  energy_flow_measure=false
      settings: InternalSimscapePortConfiguration="{\"Bottom\":[],\"Left\":[{\"id\":\"A\",\"label\":\"A\",\"type\":\"foundation.thermal_liquid.thermal_liquid\"}],\"Right\":[{\"id\":\"B\",\"label\":\"B\",\"type\":\"foundation.thermal_liquid.thermal_liquid\"},{\"id\":\"M\",\"label\":\"M\",\"type\":\"output\"}],\"Top\":[]}"
  Flow Resistance (2P) : fl_lib/Two-Phase Fluid/Elements/Flow Resistance (2P)  delta_p_nominal=0.045 MPa  mdot_nominal=m_dot kg/s  v_nominal=0 m^3/kg  area=0.01 m^2  laminar_fraction=1e-3
      settings: InternalSimscapePortConfiguration="{\"Bottom\":[],\"Left\":[{\"id\":\"A\",\"label\":\"A\",\"type\":\"foundation.two_phase_fluid.two_phase_fluid\"}],\"Right\":[{\"id\":\"B\",\"label\":\"B\",\"type\":\"foundation.two_phase_fluid.two_phase_fluid\"}],\"Top\":[]}"
  "Flow rate sensor : R32" : Subsystem
  From Spreadsheet : FromSpreadsheet  FileName=D:\Senior Project\Data\Classromm_Data.xlsx  SheetName=25-12-2025
  From13 : From  Commented=on  GotoTag=n_projector  TagVisibility=global
  From19 : From  Commented=on  GotoTag=n_people  TagVisibility=global
  From21 : From  Commented=on  GotoTag=n_laptop  TagVisibility=global
  From22 : From  Commented=on  GotoTag=n_Light  TagVisibility=global
  From24 : From  Commented=on  GotoTag=S_Water  TagVisibility=global
  From6 : From  Commented=on  GotoTag=on_off_Pump  TagVisibility=global
  Gain : Gain  Gain=0.05
  Gain1 : Gain  Commented=on  Gain=4.32
  Gain{10..12,14} (4 alike) : Gain  Gain=1/3600
  Gain13 : Gain  Gain=0.03
  Gain2 : Gain  Commented=on  Gain=2
  Gain20 : Gain  Commented=on  Gain=1.152
  Gain3 : Gain  Commented=on  Gain=13
  Gain4 : Gain  Commented=on  Gain=8
  Gain5 : Gain  Commented=on  Gain=3.6
  Gain6 : Gain  Commented=on  Gain=41
  Gain7 : Gain  Commented=on  Gain=30
  Gain8 : Gain  Gain=0.03
  Gain9 : Gain  Gain=0.84
  Goto14 : Goto  Commented=on  GotoTag=T_Tank  TagVisibility=global
  Heat Flow Rate Sensor : fl_lib/Thermal/Thermal Sensors/Heat Flow Rate Sensor
  Heat Flow Rate Sensor1 : fl_lib/Thermal/Thermal Sensors/Heat Flow Rate Sensor
  House Thermal Network : Subsystem  Tag=PublishSubsystem  mask(House Thermal Network){area_roof=35.74, thickness_roof=0.35, rho_roof=600, cp_roof=840, k_roof=0.01, hc_roof_interior=Wall_h_in, hc_roof_exterior=Wall_h_out, T_init_roof=T_Room_int_C, area_wall=(8.86+8.51)*2.6, thickness_wall=0.35, rho_wall=600, cp_wall=835, k_wall=0.007, hc_wall_interior=Wall_h_in, hc_wall_exterior=Wall_h_out, T_init_wall=T_Room_int_C, area_wall_inside=2.6*(8.86+7.31), thickness_wall_inside=0.25, rho_wall_inside=700, cp_wall_inside=650, k_wall_inside=0.004, hc_wall_inside_interior=Wall_h_in, T_init_wall_inside=T_Room_int_C, area_window=9, thickness_window=0.07, rho_window=2700, cp_window=840, k_window=0.75, hc_window_interior=25, hc_window_exterior=32, T_init_window=T_Room_int_C, area_furniture=30, M_furniture=1, cp_furniture=1500, hc_furniture_interior=18, T_init_furniture=T_Room_int_C}
      mask prompts: area_roof "Total area (m^2)"; thickness_roof "Average thickness (m)"; rho_roof "Average density (kg/m^3)"; cp_roof "Average specific heat (J/kg/K)"; k_roof "Average conductivity (W/m/K)"; hc_roof_interior "Interior heat transfer coefficient (W/m^2/K)"; hc_roof_exterior "Exterior heat transfer coefficient (W/m^2/K)"; T_init_roof "Initial temperature (degC)"; area_wall "Total area (m^2)"; thickness_wall "Average thickness (m)"; rho_wall "Average density (kg/m^3)"; cp_wall "Average specific heat (J/kg/K)"; k_wall "Average conductivity (W/m/K)"; hc_wall_interior "Interior heat transfer coefficient (W/m^2/K)"; hc_wall_exterior "Exterior heat transfer coefficient (W/m^2/K)"; T_init_wall "Initial temperature (degC)"; area_wall_inside "Total area (m^2)"; thickness_wall_inside "Average thickness (m)"; rho_wall_inside "Average density (kg/m^3)"; cp_wall_inside "Average specific heat (J/kg/K)"; k_wall_inside "Average conductivity (W/m/K)"; hc_wall_inside_interior "Interior heat transfer coefficient (W/m^2/K)"; T_init_wall_inside "Initial temperature (degC)"; area_window "Total area (m^2)"; thickness_window "Average thickness (m)"; rho_window "Average density (kg/m^3)"; cp_window "Average specific heat (J/kg/K)"; k_window "Average conductivity (W/m/K)"; hc_window_interior "Interior heat transfer coefficient (W/m^2/K)"; hc_window_exterior "Exterior heat transfer coefficient (W/m^2/K)"; T_init_window "Initial temperature (degC)"; area_furniture "Total surface area (m^2)"; M_furniture "Total mass (kg)"; cp_furniture "Average specific heat (J/kg/K)"; hc_furniture_interior "Interior heat transfer coefficient (W/m^2/K)"; T_init_furniture "Initial temperature (degC)"
      mask help: This subsystem models heat transfer between the air in the interior of the house and the external environment.
      mask DialogControl TabRoof Prompt: Roof
      mask DialogControl TabWall Prompt: Exterior Walls
      mask DialogControl TabWallInside Prompt: Interior Walls
      mask DialogControl TabWindow Prompt: Windows
      mask DialogControl TabFurniture Prompt: Furniture
  Ideal Angular Velocity Source1 : fl_lib/Mechanical/Mechanical Sources/Ideal Angular Velocity Source
  Ideal Angular Velocity Source3 : fl_lib/Mechanical/Mechanical Sources/Ideal Angular Velocity Source  Commented=on
  Inlet : Subsystem
  Integrator{,1..7} (8 alike) : Integrator
  Laptop : fl_lib/Thermal/Thermal Sources/Controlled Heat Flow Rate Source  Commented=on
  Laptop Charge : fl_lib/Thermal/Thermal Sources/Controlled Heat Flow Rate Source  Commented=on
  Lights : fl_lib/Thermal/Thermal Sources/Controlled Heat Flow Rate Source  Commented=on
  Master Valve : SimscapeFluids_lib/Thermal Liquid/Valves & Orifices/Directional Control Valves/3-Way Directional Valve (TL)  open_orifices_pos=fluids.thermal_liquid.valves.directional_control_valves.enum.OpenOrifices3Way.PA  open_orifices_neg=fluids.thermal_liquid.valves.directional_control_valves.enum.OpenOrifices3Way.AT  area_spec=fluids.thermal_liquid.valves.directional_control_valves.enum.area_spec.identical  valve_spec=fluids.thermal_liquid.valves.directional_control_valves.enum.ValveSpec.Linear  del_S_max=0.01 m  area_max=0.01 m^2  del_S_TLU=[0, .00125, .0025, .00375, .005] m  valve_area_TLU=[1e-10, 1e-05, 4e-05, 8e-05, .0001] m^2  del_S_flow_TLU=[0, .00125, .0025, .00375, .005] m  p_diff_TLU=[-.1, .3, .5, .7] MPa  vol_flow_TLU=[-9.05e-10, 1.57e-09, 2.02e-09, 2.39e-09; -9.05e-05, .000157, .000202, .000239; -.000362, .000627, .00081, .000958; -.000724, .00125, .00162, .00192; -.000905, .00156, .002, .00239] m^3/s  mdot_TLU=1e3 * [-9.05e-10, 1.57e-09, 2.02e-09, 2.39e-09; -9.05e-05, .000157, .000202, .000239; -.000362, .000627, .00081, .000958; -.000724, .00125, .00162, .00192; -.000905, .00156, .002, .00239] kg/s  T_ref_in=293.15 K  p_ref_in=0.101325 MPa  area_leak=1e-10 m^2  Cd=0.9  Re_c=150  smoothing_factor=0.01  pressure_recovery=false  area=0.015 m^2  S_max_PA=0.01 m  del_S_max_PA=0.005 m  area_max_PA=1e-4 m^2  del_S_TLU_PA=[0, .00125, .0025, .00375, .005] m  valve_area_TLU_PA=[1e-10, 1e-05, 4e-05, 8e-05, .0001] m^2  del_S_flow_TLU_PA=[0, .00125, .0025, .00375, .005] m  p_diff_TLU_PA=[-.1, .3, .5, .7] MPa  vol_flow_TLU_PA=[-9.05e-10, 1.57e-09, 2.02e-09, 2.39e-09; -9.05e-05, .000157, .000202, .000239; -.000362, .000627, .00081, .000958; -.000724, .00125, .00162, .00192; -.000905, .00156, .002, .00239] m^3/s  mdot_TLU_PA=1e3 * [-9.05e-10, 1.57e-09, 2.02e-09, 2.39e-09; -9.05e-05, .000157, .000202, .000239; -.000362, .000627, .00081, .000958; -.000724, .00125, .00162, .00192; -.000905, .00156, .002, .00239] kg/s  S_max_AT=-0.01 m  del_S_max_AT=0.005 m  area_max_AT=1e-4 m^2  del_S_TLU_AT=[0, .00125, .0025, .00375, .005] m  valve_area_TLU_AT=[1e-10, 1e-05, 4e-05, 8e-05, .0001] m^2  del_S_flow_TLU_AT=[0, .00125, .0025, .00375, .005] m  p_diff_TLU_AT=[-.1, .3, .5, .7] MPa  vol_flow_TLU_AT=[-9.05e-10, 1.57e-09, 2.02e-09, 2.39e-09; -9.05e-05, .000157, .000202, .000239; -.000362, .000627, .00081, .000958; -.000724, .00125, .00162, .00192; -.000905, .00156, .002, .00239] m^3/s  mdot_TLU_AT=1e3 * [-9.05e-10, 1.57e-09, 2.02e-09, 2.39e-09; -9.05e-05, .000157, .000202, .000239; -.000362, .000627, .00081, .000958; -.000724, .00125, .00162, .00192; -.000905, .00156, .002, .00239] kg/s  S_max_PT=4.5e-3 m  del_S_max_PT=0.005 m  area_max_PT=1e-4 m^2  del_S_TLU_PT=[0, .00125, .0025, .00375, .005] m  valve_area_TLU_PT=[1e-10, 1e-05, 4e-05, 8e-05, .0001] m^2  del_S_flow_TLU_PT=[0, .00125, .0025, .00375, .005] m  p_diff_TLU_PT=[-.1, .3, .5, .7] MPa  vol_flow_TLU_PT=[-9.05e-10, 1.57e-09, 2.02e-09, 2.39e-09; -9.05e-05, .000157, .000202, .000239; -.000362, .000627, .00081, .000958; -.000724, .00125, .00162, .00192; -.000905, .00156, .002, .00239] m^3/s  mdot_TLU_PT=1e3 * [-9.05e-10, 1.57e-09, 2.02e-09, 2.39e-09; -9.05e-05, .000157, .000202, .000239; -.000362, .000627, .00081, .000958; -.000724, .00125, .00162, .00192; -.000905, .00156, .002, .00239] kg/s
      settings: InternalSimscapePortConfiguration="{\"Bottom\":[],\"Left\":[{\"id\":\"A\",\"label\":\"A\",\"type\":\"foundation.thermal_liquid.thermal_liquid\"}],\"Right\":[{\"id\":\"S\",\"label\":\"S\",\"type\":\"input\"},{\"id\":\"P\",\"label\":\"P\",\"type\":\"foundation.thermal_liquid.thermal_liquid\"},{\"id\":\"T\",\"label\":\"T\",\"type\":\"foundation.thermal_liquid.thermal_liquid\"}],\"Top\":[]}"
  Mechanical Rotational Reference1 : fl_lib/Mechanical/Rotational Elements/Mechanical Rotational Reference
  Mechanical Rotational Reference3 : fl_lib/Mechanical/Rotational Elements/Mechanical Rotational Reference  Commented=on
  Moist Air Properties (MA)2 : fl_lib/Moist Air/Utilities/Moist Air Properties (MA)  R_a=287.047 J/(K*kg)  T_TLU=[-56.55, -50 : 10 : -10, -5 : 1 : 5, 10 : 10 : 350]' degC  h_a_TLU=[342.414066793634; 349.003411914139; 359.061417476782; 369.117728274935; 379.173188407993; 389.228602960013; 394.256538873206; 395.262156814682; 396.26778682262; 397.27342967397; 398.279086145689; 399.284757014822; 400.290443058569; 401.296145054364; 402.301863779931; 403.307600013352; 404.313354533128; 409.342428711098; 419.402397945314; 429.465451846544; 439.532387826623; 449.604014793745; 459.68115297076; 469.764632657687; 479.855292205971; 489.953975419749; 500.06152856014; 510.178797098051; 520.306622336267; 530.445838000969; 540.597266885076; 550.761717610289; 560.939981561004; 571.132830031086; 581.341011613777; 591.565249855533; 601.806241186423; 612.064653132654; 622.341122810862; 632.636255698901; 642.95062467384; 653.284769304793; 663.639195385783; 674.014374692179; 684.410744943084; 694.828709951456; 705.268639943519; 715.730872029167; 726.215710805484; 736.723429076127; 747.254268670154; 757.808441344776] kJ/kg  mu_a_TLU=[14.2568884161326; 14.6140128551699; 15.151727785151; 15.6806860927178; 16.201235181264; 16.7137043838401; 16.9670072430524; 17.017438132541; 17.0677931537044; 17.1180726001803; 17.1682767640582; 17.2184059358881; 17.2684604046898; 17.318440457962; 17.3683463816913; 17.4181784603614; 17.467936976962; 17.7156359301048; 18.2056752419787; 18.6887904184394; 19.1652345249932; 19.6352479488881; 20.099059157425; 20.5568854116507; 21.008933436444; 21.4554000485251; 21.8964727442509; 22.3323302492491; 22.7631430320408; 23.1890737838183; 23.6102778665211; 24.0269037312887; 24.4390933092858; 24.8469823767971; 25.2507008963847; 25.6503733357905; 26.0461189661617; 26.438052141067; 26.8262825576728; 27.210915501349; 27.5920520748824; 27.969789413389; 28.3442208859359; 28.7154362848061; 29.0835220032714; 29.4485612026716; 29.8106339695395; 30.169817463453; 30.5261860562487; 30.8798114631771; 31.2307628665438; 31.5791070323335] s*uPa  k_a_TLU=[19.8808491891482; 20.4162457047568; 21.2248745869044; 22.0232455041378; 22.8117316528767; 23.59069155438; 23.9767077285082; 24.0536401764626; 24.130482853517; 24.2072360894785; 24.2839002127411; 24.3604755502875; 24.4369624276914; 24.5133611691197; 24.5896720973349; 24.6658955336975; 24.7420317981691; 25.1214166432482; 25.8738284673185; 26.6180151791963; 27.3542675863918; 28.0828636150405; 28.8040688184917; 29.5181369069754; 30.2253102842368; 30.9258205811167; 31.6198891790667; 32.307727718801; 32.989538590917; 33.6655154065126; 34.3358434467079; 35.0007000906151; 35.6602552217624; 36.314671613305; 36.9641052925838; 37.6087058857479; 38.2486169432557; 38.8839762471259; 39.5149161008418; 40.1415636028127; 40.7640409042923; 41.3824654526272; 41.9969502206863; 42.6076039232795; 43.2145312213471; 43.8178329146528; 44.4176061236819; 45.0139444614019; 45.6069381955058; 46.1966744017242; 46.7832371087507; 47.3667074352967] mW/(K*m)  p_min=1 kPa  p_max=inf MPa  T_min=-56.55 degC  T_max=350 degC  properties_range_check=simscape.enum.assert.action.error  p_atm=0.101325 MPa  T_atm=20 degC  enable_droplets=false  R_w=461.523 J/(K*kg)  p_ws_TLU=[1.71168953425982e-06; 3.93770601979424e-06; 1.28411717710344e-05; 3.80051394873809e-05; .00010323902900209; .000259873810798063; .000401741022116384; .000437454836117844; .000476040820618202; .000517704666185737; .000562664883741207; .000611212677444345; .000657085634113763; .000705985593917791; .00075808051438111; .000813548355379396; .000872575113841924; .00122819910164487; .00233931836947519; .00424697076171126; .00738493802968097; .012351945812707; .0199464343236764; .0312009300307261; .0474144740241604; .0701817658485933; .101417996663294; .143378712947169; .198674420476403; .270279976781692; .361539099388177; .476164537971214; .618234621423587; .792187006980199; 1.00281053608169; 1.25523615516845; 1.55492790046272; 1.90767499353199; 2.31958617020155; 2.79708749692822; 3.34692514426746; 3.97617493064794; 4.69226099229504; 5.50298678300951; 6.41658290952841; 7.44177834442093; 8.58790494083256; 9.86505121117553; 11.284292927457; 12.8580516000122; 14.6006773719404; 16.5294151389953] MPa  h_w_vap_TLU=[2836.88241275372; 2837.81392500514; 2838.63937175807; 2838.7309929628; 2838.06905313927; 2836.62597341095; 2835.60023952573; 2835.37006381376; 2835.13143158077; 2834.88429145066; 2834.62859062897; 2500.93420564316; 2498.55452890293; 2496.17317793437; 2493.7941260618; 2491.41713708944; 2489.04199020767; 2477.18706302224; 2453.51925941961; 2429.81122987564; 2405.97728678685; 2381.94712654051; 2357.65452030374; 2333.03120800924; 2308.00352809267; 2282.49062771796; 2256.40372152657; 2229.64615315163; 2202.11407337172; 2173.6974807639; 2144.28128268553; 2113.74600964951; 2081.9678834089; 2048.81807129851; 2014.16109962579; 1977.85249331179; 1939.73572816654; 1899.63852389863; 1857.36838273035; 1812.70710332357; 1765.4037880462; 1715.16561416478; 1661.64526339623; 1604.4232249434; 1542.98206457018; 1476.66790089115; 1404.63083498414; 1325.72875296442; 1238.36212284382; 1140.16281350074; 1027.31658328826; 892.746804215825] kJ/kg  h_w_TLU=[2396.53078650168; 2408.65722023252; 2427.16766028467; 2445.66624034104; 2464.1379798878; 2482.5594701893; 2491.7412703989; 2493.57467660537; 2495.40699233755; 2497.23816944599; 2499.06815833272; 2500.89261781717; 2502.73123919979; 2504.56496564907; 2506.39800457704; 2508.23033644628; 2510.06194120626; 2519.20831890725; 2537.43340437276; 2555.54520329515; 2573.51032237465; 2591.28888786817; 2608.83487221908; 2626.09640083333; 2643.01588134754; 2659.53001419864; 2675.5827869577; 2696.18462565746; 2716.49989554204; 2736.6235211014; 2756.61216047677; 2776.50561774616; 2796.33378923373; 2816.11979584021; 2835.88181424959; 2855.6343057571; 2875.38889328914; 2895.15500578618; 2914.94035966265; 2934.75132291939; 2954.59319332093; 2974.47041287496; 2994.38673461102; 3014.34535330297; 3034.34900869544; 3054.40006758361; 3074.50058949656; 3094.65237956705; 3114.85703131193; 3135.11596141057; 3155.43043809331; 3175.80160439414] kJ/kg  mu_w_TLU=[6.9886414857741; 7.21462000349698; 7.55962537406626; 7.90463074463554; 8.24963611520482; 8.5946414857741; 8.76714417105874; 8.80164470811567; 8.8361452451726; 8.87064578222952; 8.90514631928645; 8.93964685634338; 8.97414739340031; 9.00294911497154; 9.0318980288863; 9.06099135942002; 9.09022638806001; 9.23843559844524; 9.5440595677542; 9.86015858692705; 10.1848429274122; 10.5164578096049; 10.8535319382781; 11.1947482575333; 11.5389294976352; 11.8850331780701; 12.2322493177351; 12.6188533568459; 13.0082793358938; 13.4003380262893; 13.7948421428098; 14.1916095618232; 14.590464747099; 14.9912394314964; 15.3937729006119; 15.7979120385447; 16.203511226482; 16.610432150303; 17.0185435533718; 17.4277209582061; 17.8378463726577; 18.2488079909412; 18.6604998963166; 19.0728217698535; 19.485678608085; 19.8989804512625; 20.3126421231677; 20.7265829829225; 21.1407266888906; 21.5550009745266; 21.969337435876; 22.3836713303269] s*uPa  k_w_TLU=[12.4916816538045; 12.9847788176262; 13.737598915064; 14.4904190125018; 15.2432391099396; 15.9960592073774; 16.3724692560963; 16.4477512658401; 16.5230332755839; 16.5983152853277; 16.6735972950715; 16.7488793048152; 16.824161314559; 16.8886088206517; 16.9532779906513; 17.0181691764255; 17.083282769915; 17.4122036181723; 18.0870861656185; 18.7855813517187; 19.5093466408385; 20.2607864040347; 21.0430876297671; 21.8602068151121; 22.7168164077153; 23.6182141540994; 24.5698636875305; 25.4024944426483; 26.2458938647479; 27.1009155051916; 27.968142896353; 28.8479507975112; 29.7405485790829; 30.646029672269; 31.5643932662527; 32.4955693285114; 33.4394360046859; 34.3958329885356; 35.3645718140131; 36.3454437886179; 37.3382261129791; 38.3426866012072; 39.3585873185985; 40.3856873794121; 41.4237450915028; 42.4725195920623; 43.5317720862424; 44.6012667755489; 45.6807715437344; 46.7700584531355; 47.8689040929333; 48.9770898119082] mW/(K*m)  D_w=25 mm^2/s  trace_gas_model=foundation.enum.trace_gas_model.none  R_g=188.923 J/(K*kg)  h_g_TLU=[439.555216276024; 444.670268214299; 452.538618857965; 460.487124266174; 468.522588773143; 476.64941595933; 480.747985385885; 481.570543185868; 482.394052396612; 483.218514286302; 484.043930026094; 484.87030069324; 485.697627274149; 486.525910667382; 487.355151686572; 488.185351063277; 489.016509449741; 493.186704132078; 501.599194941473; 510.107689945701; 518.711611059603; 527.410026767716; 536.20176474847; 545.085474167968; 554.059675464379; 563.122805439004; 572.273250917104; 581.509372969931; 590.829525041787; 600.232066635428; 609.715373504524; 619.277845094572; 628.91790983254; 638.634028741375; 648.424697754692; 658.288449028076; 668.22385148184; 678.229510761734; 688.30406876583; 698.446202855373; 708.654624842952; 718.928079831753; 729.265344963773; 739.665228122078; 750.126566621791; 760.648225916092; 771.229098336723; 781.86810188302; 792.564179069104; 803.316295835373; 814.123440527678; 824.984622945405] kJ/kg  mu_g_TLU=[10.9386626034033; 11.2618160869372; 11.7542862475187; 12.2454955799777; 12.7352208796158; 13.2232325321233; 13.4665248390743; 13.5151226761166; 13.5636997995993; 13.6122559954699; 13.6607910510226; 13.709304754931; 13.757796897279; 13.8062672695897; 13.8547156648526; 13.9031418775498; 13.9515457036801; 14.1932220047332; 14.6747828595747; 15.153802214283; 15.6301123398299; 16.1035631756244; 16.574022106427; 17.0413733976215; 17.5055174102327; 17.9663696812767; 18.4238599299346; 18.8779310322956; 19.3285379947687; 19.7756469471288; 20.2192341695255; 20.6592851629269; 21.0957937689132; 21.5287613421341; 21.9581959768344; 22.3841117874779; 22.8065282425078; 23.2254695495877; 23.6409640901974; 24.0530439011453; 24.4617442003854; 24.8671029544344; 25.269160484669; 25.6679591098169; 26.0635428220247; 26.4559569939835; 26.8452481147025; 27.2314635516519; 27.6146513371198; 27.9948599767665; 28.3721382784874; 28.74653519983] s*uPa  k_g_TLU=[10.7373095949238; 11.1772934980884; 11.862915506018; 12.5638333280734; 13.2785475592421; 14.005722199619; 14.3736017704762; 14.4475028211958; 14.5215096973787; 14.5956213250986; 14.6698366403414; 14.7441545888563; 14.8185741260114; 14.8930942166532; 14.9677138349692; 15.0424319643548; 15.1172475972825; 15.4927536712633; 16.2505237772467; 17.0165521650722; 17.7899991951805; 18.5700903932503; 19.3561099002839; 20.1473949639617; 20.9433312278214; 21.7433486448307; 22.5469178892132; 23.3535471729555; 24.1627793965491; 24.9741895799701; 25.7873825314493; 26.6019907190427; 27.4176723115859; 28.2341093347412; 29.0510055857402; 29.8680879651392; 30.6851034165693; 31.5018116707882; 32.3179924018673; 33.1334410491403; 33.9479677779769; 34.7613965127281; 35.5735640361829; 36.3843191504339; 37.1935218945334; 38.0010428147395; 38.80676228352; 39.6105698638057; 40.412363715274; 41.2120500397018; 42.0095425626597; 42.8047620490288] mW/(K*m)  D_g=16 mm^2/s
  Mux : Mux  Inputs=3'
  Mux{1,3,5..6} (4 alike) : Mux  Inputs=2
  Mux2 : Mux  Inputs=6
  Mux4 : Mux  Inputs=3
  Mux7 : Mux  Inputs=3
  Mux8 : Mux  Inputs=3
  Occupants : fl_lib/Thermal/Thermal Sources/Controlled Heat Flow Rate Source  Commented=on
  Outlet : Subsystem
      settings: PortSchema="{\"entries\":[{\"content\":{\"sides\":[{\"content\":{},\"type\":\"ConnectorPlacement.EquallySpacedRectSide\",\"uuid\":\"c21d58b1-84ae-41b5-8457-01953e7a09e4\"},{\"content\":{\"side\":\"RIGHT\"},\"type\":\"ConnectorPlacement.EquallySpacedRectSide\",\"uuid\":\"aa3b7831-58c0-4bcb-9fdb-1ced2b8fb954\"},{\"content\":{\"connectorIds\":[\"LConn1\"],\"side\":\"TOP\"},\"type\":\"ConnectorPlacement.EquallySpacedRectSide\",\"uuid\":\"eaa7610a-31aa-44a1-9e24-e280e426f208\"}]},\"type\":\"ConnectorPlacement.EquallySpacedConnector\",\"uuid\":\"7a098441-fec4-4e5c-a8c2-a976ae9fb3d4\"}],\"packageUris\":[\"http://schema.mathworks.com/mf0/Connector/R2020b\"],\"version\":\"1.0\"}"
  PS Gain1 : fl_lib/Physical Signals/Functions/PS Gain  Commented=on  gain=500 rpm
  PS Gain2 : fl_lib/Physical Signals/Functions/PS Gain  gain=500 rpm
  PS-Simulink Converter{,1,3,6,8} (5 alike) : nesl_utility/PS-Simulink Converter  PhysicalDomain=network_engine_domain  SubClassName=ps_output  LeftPortType=input  RightPortType=output  PseudoPeriodic=off  Frequencies=[]  VectorFormat=inherit  Unit=kW  AffineConversion=on
  PS-Simulink Converter10 : nesl_utility/PS-Simulink Converter  PhysicalDomain=network_engine_domain  SubClassName=ps_output  LeftPortType=input  RightPortType=output  PseudoPeriodic=off  Frequencies=[]  VectorFormat=inherit  Unit=1  AffineConversion=off
  PS-Simulink Converter{4,11..13} (4 alike) : nesl_utility/PS-Simulink Converter  PhysicalDomain=network_engine_domain  SubClassName=ps_output  LeftPortType=input  RightPortType=output  PseudoPeriodic=off  Frequencies=[]  VectorFormat=inherit  Unit=degC  AffineConversion=on
  PS-Simulink Converter2 : nesl_utility/PS-Simulink Converter  Commented=on  PhysicalDomain=network_engine_domain  SubClassName=ps_output  LeftPortType=input  RightPortType=output  PseudoPeriodic=off  Frequencies=[]  VectorFormat=inherit  Unit=degC  AffineConversion=on
  PS-Simulink Converter5 : nesl_utility/PS-Simulink Converter  PhysicalDomain=network_engine_domain  SubClassName=ps_output  LeftPortType=input  RightPortType=output  PseudoPeriodic=off  Frequencies=[]  VectorFormat=inherit  Unit=inherit  AffineConversion=off
  PS-Simulink Converter7 : nesl_utility/PS-Simulink Converter  PhysicalDomain=network_engine_domain  SubClassName=ps_output  LeftPortType=input  RightPortType=output  PseudoPeriodic=off  Frequencies=[]  VectorFormat=inherit  Unit=1  AffineConversion=off
  PS-Simulink Converter9 : nesl_utility/PS-Simulink Converter  PhysicalDomain=network_engine_domain  SubClassName=ps_output  LeftPortType=input  RightPortType=output  PseudoPeriodic=off  Frequencies=[]  VectorFormat=inherit  Unit=1  AffineConversion=off
  Pipe (TL)1 : fl_lib/Thermal Liquid/Elements/Pipe (TL)  length=5 m  area=0.01 m^2  Dh=0.1128 m  length_add=1 m  roughness=15e-6 m  Re_lam=2000  Re_tur=4000  shape_factor=64  Nu_lam=3.66  dynamic_compressibility=true  inertia=false  p0=0.101325 MPa  T0=293.15 K  mdot0=0 kg/s  p_nominal=0.101325 MPa  T_nominal=293.15 K
  Pipe (TL)2 : fl_lib/Thermal Liquid/Elements/Pipe (TL)  length=5 m  area=0.01 m^2  Dh=0.1128 m  length_add=1 m  roughness=15e-6 m  Re_lam=2000  Re_tur=4000  shape_factor=64  Nu_lam=3.66  dynamic_compressibility=true  inertia=false  p0=0.101325 MPa  T0=293.15 K  mdot0=0 kg/s  p_nominal=0.101325 MPa  T_nominal=293.15 K
  Pipe (TL)3 : fl_lib/Thermal Liquid/Elements/Pipe (TL)  Commented=on  length=1 m  area=0.03*0.03*pi m^2  Dh=0.03*2*pi m  length_add=1 m  roughness=15e-6 m  Re_lam=2000  Re_tur=4000  shape_factor=64  Nu_lam=3.66  dynamic_compressibility=true  inertia=false  p0=0.101325 MPa  T0=T_Tank_int_c degC  mdot0=0 kg/s  p_nominal=0.101325 MPa  T_nominal=293.15 K
  Pipe (TL)4 : fl_lib/Thermal Liquid/Elements/Pipe (TL)  Commented=on  length=0.1 m  area=0.03*0.03*pi m^2  Dh=2*0.03*pi m  length_add=1 m  roughness=15e-6 m  Re_lam=2000  Re_tur=4000  shape_factor=64  Nu_lam=3.66  dynamic_compressibility=true  inertia=false  p0=0.101325 MPa  T0=T_Tank_int_c degC  mdot0=0 kg/s  p_nominal=0.101325 MPa  T_nominal=293.15 K
  Pipe (TL)5 : fl_lib/Thermal Liquid/Elements/Pipe (TL)  Commented=on  length=1 m  area=0.03*0.03*pi m^2  Dh=0.03*2*pi m  length_add=1 m  roughness=15e-6 m  Re_lam=2000  Re_tur=4000  shape_factor=64  Nu_lam=3.66  dynamic_compressibility=true  inertia=false  p0=0.101325 MPa  T0=T_Tank_int_c degC  mdot0=0 kg/s  p_nominal=0.101325 MPa  T_nominal=293.15 K
  Positive-Displacement Compressor (2P) : SimscapeFluids_lib/Two-Phase Fluid/Fluid Machines/Positive-Displacement Compressor (2P)  dispSpec=fluids.two_phase_fluid.fluid_machines.enum.DisplacementSpecification.Displacement  v_disp=34 cm^3/rev  mdot_nom=0.01 kg/s  omega_nom=1000 rpm  efficiencySpec=fluids.two_phase_fluid.fluid_machines.enum.VolumetricEfficiencyParameterization.Analytical  thermodynamicModelSpec=fluids.two_phase_fluid.fluid_machines.enum.ThermodynamicModel.Polytropic  n=1.165  eta_isen=0.65  eta_isen_TLU=[.95, .9, .85, .8, .75; .925, .875, .825, .775, .725; .875, .825, .775, .725, .675; .75, .7, .65, .6, .55]  eta_vol_nom=0.95  pr_TLU=[2, 4, 6, 8]  omega_TLU=[800, 1500, 2800, 3300, 4000] rpm  eta_vol_TLU=[.95, .9, .85, .8, .75; .925, .875, .825, .775, .725; .875, .825, .775, .725, .675; .75, .7, .65, .6, .55]  nominalSpec=fluids.two_phase_fluid.fluid_machines.enum.NominalConditionsSpecification.Pressure  pr_nom=P2/P1  p_in_nom=0.101325 MPa  T_in_nom=373.15 K  T_evap_nom=373.15 K  T_cond_nom=398.15 K  delta_T_nom=10 deltaK  mechanical_efficiency=0.9  area_A=0.01 m^2  area_B=0.01 m^2  VaporCheck=simscape.enum.assert.action.none
      settings: InternalSimscapePortConfiguration="{\"Bottom\":[],\"Left\":[{\"id\":\"A\",\"label\":\"A\",\"type\":\"foundation.two_phase_fluid.two_phase_fluid\"},{\"id\":\"C\",\"label\":\"C\",\"type\":\"foundation.mechanical.rotational.rotational\"}],\"Right\":[{\"id\":\"B\",\"label\":\"B\",\"type\":\"foundation.two_phase_fluid.two_phase_fluid\"},{\"id\":\"R\",\"label\":\"R\",\"type\":\"foundation.mechanical.rotational.rotational\"}],\"Top\":[]}"
  Pressure & Temperature Sensor (MA) : fl_lib/Moist Air/Sensors/Pressure & Temperature Sensor (MA)  reference=foundation.enum.MeasurementReference.absolute  pressure=false  pressure_spec=foundation.enum.PressureMeasementSpec.Absolute  temperature=true
      settings: InternalSimscapePortConfiguration="{\"Bottom\":[{\"id\":\"T\",\"label\":\"T\",\"type\":\"output\"}],\"Left\":[{\"id\":\"A\",\"label\":\"A\",\"type\":\"foundation.moist_air.moist_air\"}],\"Right\":[],\"Top\":[]}"
  Pressure & Temperature Sensor (MA)1 : fl_lib/Moist Air/Sensors/Pressure & Temperature Sensor (MA)  reference=foundation.enum.MeasurementReference.absolute  pressure=false  pressure_spec=foundation.enum.PressureMeasementSpec.Absolute  temperature=true
      settings: InternalSimscapePortConfiguration="{\"Bottom\":[{\"id\":\"T\",\"label\":\"T\",\"type\":\"output\"}],\"Left\":[{\"id\":\"A\",\"label\":\"A\",\"type\":\"foundation.moist_air.moist_air\"}],\"Right\":[],\"Top\":[]}"
  Projector : fl_lib/Thermal/Thermal Sources/Controlled Heat Flow Rate Source  Commented=on
  Q_Charge : Subsystem
  Q_Charge1 : Subsystem
  R32 : SimscapeFluids_lib/Two-Phase Fluid/Utilities/Two-Phase Fluid Predefined Properties (2P)  fluid=fluids.two_phase_fluid.utilities.enum.Fluid.R32  p_atm=0.101325 MPa  properties_range_check=simscape.enum.assert.action.error  q_rev=0.01 Pa
  Receiver Accumulator (2P) : SimscapeFluids_lib/Two-Phase Fluid/Tanks & Accumulators/Receiver Accumulator (2P)  volume=1 m^3  tank_area=0.5 m^2  area_AV=0.01 m^2  area_BV=0.01 m^2  area_AL=0.01 m^2  area_BL=0.01 m^2  V_frac_liq_error=simscape.enum.assert.action.none  V_frac_liq_min=0.05  V_frac_liq_max=0.95  V_frac_smooth=0.05  p_crit_error=simscape.enum.assert.action.error  hc_vap=20 W/(K*m^2)  hc_liq=100 W/(K*m^2)  p_init=P3-0.045 MPa  fraction_spec=fluids.two_phase_fluid.tanks_accumulators.enum.LiquidFractionSpec.Volume  M_frac_liq_init=0.5  V_frac_liq_init=0.5  saturated_init=true  energy_spec=fluids.two_phase_fluid.tanks_accumulators.enum.EnergySpec.SubcoolingSuperheating  delta_T_sub_init=5 deltaK  delta_T_sup_init=5 deltaK  T_liq_init=368.15 K  T_vap_init=378.15 K  h_liq_init=400 kJ/kg  h_vap_init=2700 kJ/kg  u_liq_init=400 kJ/kg  u_vap_init=2700 kJ/kg  tau_vap_cond=0.1 s
      settings: InternalSimscapePortConfiguration="{\"Bottom\":[],\"Left\":[{\"id\":\"AV\",\"label\":\"AV\",\"type\":\"foundation.two_phase_fluid.two_phase_fluid\"},{\"id\":\"AL\",\"label\":\"AL\",\"type\":\"foundation.two_phase_fluid.two_phase_fluid\"},{\"id\":\"H\",\"label\":\"H\",\"type\":\"foundation.thermal.thermal\"}],\"Right\":[{\"id\":\"BV\",\"label\":\"BV\",\"type\":\"foundation.two_phase_fluid.two_phase_fluid\"},{\"id\":\"BL\",\"label\":\"BL\",\"type\":\"foundation.two_phase_fluid.two_phase_fluid\"},{\"id\":\"L\",\"label\":\"L\",\"type\":\"output\"}],\"Top\":[]}"
  Relay : Relay  Commented=on  OnSwitchValue=1  OffSwitchValue=-1  OnOutputValue=0  OffOutputValue=1
  S1 : Subsystem
  S2 : Subsystem
  S3 : Subsystem
  S4 : Subsystem
      settings: PortSchema="{\"entries\":[{\"content\":{\"sides\":[{\"content\":{},\"type\":\"ConnectorPlacement.EquallySpacedRectSide\",\"uuid\":\"744b6a87-1fb4-4e0c-8c4c-5d04732f137d\"},{\"content\":{\"side\":\"RIGHT\"},\"type\":\"ConnectorPlacement.EquallySpacedRectSide\",\"uuid\":\"713931cd-e0c1-496d-ab4f-25c701c5222a\"},{\"content\":{\"connectorIds\":[\"LConn1\"],\"side\":\"TOP\"},\"type\":\"ConnectorPlacement.EquallySpacedRectSide\",\"uuid\":\"f06713a3-8a20-49e0-b549-a4ea79622a2e\"}]},\"type\":\"ConnectorPlacement.EquallySpacedConnector\",\"uuid\":\"f890a01f-659c-4927-9b37-968cf0ae8758\"}],\"packageUris\":[\"http://schema.mathworks.com/mf0/Connector/R2020b\"],\"version\":\"1.0\"}"
  S5 : Subsystem
      settings: PortSchema="{\"entries\":[{\"content\":{\"sides\":[{\"content\":{},\"type\":\"ConnectorPlacement.EquallySpacedRectSide\",\"uuid\":\"744b6a87-1fb4-4e0c-8c4c-5d04732f137d\"},{\"content\":{\"side\":\"RIGHT\"},\"type\":\"ConnectorPlacement.EquallySpacedRectSide\",\"uuid\":\"713931cd-e0c1-496d-ab4f-25c701c5222a\"},{\"content\":{\"connectorIds\":[\"LConn1\"],\"side\":\"TOP\"},\"type\":\"ConnectorPlacement.EquallySpacedRectSide\",\"uuid\":\"f06713a3-8a20-49e0-b549-a4ea79622a2e\"}]},\"type\":\"ConnectorPlacement.EquallySpacedConnector\",\"uuid\":\"f890a01f-659c-4927-9b37-968cf0ae8758\"}],\"packageUris\":[\"http://schema.mathworks.com/mf0/Connector/R2020b\"],\"version\":\"1.0\"}"
  Saturation : Saturate  UpperLimit=1  LowerLimit=0
  Scope : Scope  NumInputPorts=9
      settings: ActiveDisplayYMinimum=-0.0019412586641635282  ActiveDisplayYMaximum=0.017471327977471758
  Simulink-PS Converter : nesl_utility/Simulink-PS Converter  Commented=on  PhysicalDomain=network_engine_domain  SubClassName=ps_input  LeftPortType=input  RightPortType=output  PseudoPeriodic=off  Frequencies=[]  NoiseDistribution=none  NoiseParameters=[]  Unit=1  AffineConversion=off  FilteringAndDerivatives=provide  SimscapeFilterOrder=1  InputFilterTimeConstant=0.001  UdotUserProvided=0
  Simulink-PS Converter{1,4..6,8,10} (6 alike) : nesl_utility/Simulink-PS Converter  Commented=on  PhysicalDomain=network_engine_domain  SubClassName=ps_input  LeftPortType=input  RightPortType=output  PseudoPeriodic=off  Frequencies=[]  NoiseDistribution=none  NoiseParameters=[]  Unit=1  AffineConversion=on  FilteringAndDerivatives=provide  SimscapeFilterOrder=1  InputFilterTimeConstant=0.001  UdotUserProvided=0
  Simulink-PS Converter2 : nesl_utility/Simulink-PS Converter  Commented=on  PhysicalDomain=network_engine_domain  SubClassName=ps_input  LeftPortType=input  RightPortType=output  PseudoPeriodic=off  Frequencies=[]  NoiseDistribution=none  NoiseParameters=[]  Unit=1  AffineConversion=off  FilteringAndDerivatives=provide  SimscapeFilterOrder=1  InputFilterTimeConstant=0.001  UdotUserProvided=0
  Simulink-PS Converter3 : nesl_utility/Simulink-PS Converter  PhysicalDomain=network_engine_domain  SubClassName=ps_input  LeftPortType=input  RightPortType=output  PseudoPeriodic=off  Frequencies=[]  NoiseDistribution=none  NoiseParameters=[]  Unit=1  AffineConversion=off  FilteringAndDerivatives=provide  SimscapeFilterOrder=1  InputFilterTimeConstant=0.001  UdotUserProvided=0
  Simulink-PS Converter7 : nesl_utility/Simulink-PS Converter  PhysicalDomain=network_engine_domain  SubClassName=ps_input  LeftPortType=input  RightPortType=output  PseudoPeriodic=off  Frequencies=[]  NoiseDistribution=none  NoiseParameters=[]  Unit=1  AffineConversion=off  FilteringAndDerivatives=provide  SimscapeFilterOrder=1  InputFilterTimeConstant=0.001  UdotUserProvided=0
  Simulink-PS Converter9 : nesl_utility/Simulink-PS Converter  PhysicalDomain=network_engine_domain  SubClassName=ps_input  LeftPortType=input  RightPortType=output  PseudoPeriodic=off  Frequencies=[]  NoiseDistribution=none  NoiseParameters=[]  Unit=1  AffineConversion=off  FilteringAndDerivatives=provide  SimscapeFilterOrder=1  InputFilterTimeConstant=0.001  UdotUserProvided=0
  Solver Configuration : nesl_utility/Solver Configuration  PhysicalDomain=network_engine_domain  SubClassName=solver  LeftPortType=input  RightPortType=generic  Tones=[]  Harmonics=[]  SimulateNoise=off  Profile=off  UseLocalSampling=off  EnableSwitchedLinearOptims=on  FrequencyDomain=off  UseCCode=off  RelTol=0.001  AbsTol=0.001  MinStep=1e-09  ToWorkspace=off  RevertToSquareIcSolve=off  NumHomotopyIterations=100  PhasorMode=off  PhasorModeNumHarmonics=1  ConsistencySolver=NEWTON_XTOL_AFTER_FTOL  IndexReductionMethod=DerivativeReplacement  DoDC=off  ResidualTolerance=1e-09  ConsistencyTolSource=GLOBAL  ConsistencyAbsTol=0.001  ConsistencyRelTol=0.001  ConsistencyTolFactor=0.001  UseLocalSolver=off  LocalSolverChoice=NE_BACKWARD_EULER_ADVANCER  ResolveIndetEquations=on  FunctionEvalNumThread=1  LocalSolverSampleTime=0.001  DoFixedCost=off  MaxNonlinIter=3  MaxModeIter=2  ComputeImpulses=off  ImpulseIterations=2  LinearAlgebra=auto  LinearAlgebraNumThread=0  EquationFormulation=NE_TIME_EF  DelaysMemoryBudget=1024  AutomaticFiltering=on  FilteringTimeConstant=0.001  PartitionStorageMethod=AS_NEEDED  PartitionMemoryBudget=1024  PartitionMethod=ROBUST  MultibodyUseLocalSolver=off  MultibodyLocalSolverChoice=ODE1  MultibodyLocalSolverSampleTime=0.001
  Subsystem : Subsystem
      settings: PortSchema="{\"entries\":[{\"content\":{\"sides\":[{\"content\":{\"connectorIds\":[\"LConn1\"]},\"type\":\"ConnectorPlacement.EquallySpacedRectSide\",\"uuid\":\"36ac3938-e254-461a-ab10-353e6e8da680\"},{\"content\":{\"side\":\"RIGHT\"},\"type\":\"ConnectorPlacement.EquallySpacedRectSide\",\"uuid\":\"8ea829be-ff5f-4b21-9849-f997d1b2e55a\"},{\"content\":{\"connectorIds\":[\"LConn2\"],\"side\":\"TOP\"},\"type\":\"ConnectorPlacement.EquallySpacedRectSide\",\"uuid\":\"43605454-d5a3-4b0d-85b3-28d0e4093b39\"},{\"content\":{\"connectorIds\":[\"RConn1\"],\"side\":\"BOTTOM\"},\"type\":\"ConnectorPlacement.EquallySpacedRectSide\",\"uuid\":\"501e8f69-7fd6-4fed-a1ed-68512e4f2d0c\"}]},\"type\":\"ConnectorPlacement.EquallySpacedConnector\",\"uuid\":\"fdd5ac69-0cf2-4bbf-9fa5-10eb4260ce29\"}],\"packageUris\":[\"http://schema.mathworks.com/mf0/Connector/R2020b\"],\"version\":\"1.0\"}"
  Subsystem1 : Subsystem
  Subsystem2 : Subsystem  Commented=on
  Subsystem3 : Subsystem
  System-Level Condenser Evaporator (2P-TL) : SimscapeFluids_lib/Heat Exchangers/Two-Phase Fluid - Thermal Liquid/System-Level Condenser Evaporator (2P-TL)  flow_arrangement=fluids.heat_exchangers.enum.SystemLevelFlowArrangement2PTL.Counter  wall_thermal_mass=false  mass_wall=1 kg  cp_wall=490 J/(K*kg)  nominal_init_wall=true  T_wall_init=293.15 K  area_A1=0.01 m^2  area_B1=0.01 m^2  area_A2=0.01 m^2  area_B2=0.01 m^2  operating_condition_2P=fluids.heat_exchangers.enum.SystemLevelOperatingCondition2PTL.Evaporator  mdot_nominal_2P=m_dot kg/s  delta_p_nominal_2P=0.03 MPa  pressure_spec_cond_2P=fluids.heat_exchangers.enum.SystemLevelPressureSpecCondenser2P.InletPressure  pressure_spec_evap_2P=fluids.heat_exchangers.enum.SystemLevelPressureSpecEvaporator2P.InletPressure  p_in_nominal_2P=P4 MPa  T_cond_nominal_2P=313.15 K  T_evap_nominal_2P=243.15 K  inlet_spec_2P=fluids.heat_exchangers.enum.SystemLevelInletSpec2P.Enthalpy  T_in_nominal_2P=333.15 K  h_in_nominal_2P=h4 kJ/kg  x_in_nominal_2P=1  capacity_spec_2P=fluids.heat_exchangers.enum.SystemLevelCapacitySpec.HeatTransfer  Q_nominal=3 kW  outlet_spec_cond_2P=fluids.heat_exchangers.enum.SystemLevelOutletSpecCondenser2P.Enthalpy  outlet_spec_evap_2P=fluids.heat_exchangers.enum.SystemLevelOutletSpecEvaporator2P.Enthalpy  delta_T_sub_nominal_2P=5 deltaK  delta_T_sup_nominal_2P=5 deltaK  h_out_nominal_2P=250 kJ/kg  x_out_nominal_2P=0  volume_2P=0.001 m^3  nominal_init_2P=true  energy_spec_2P=foundation.enum.energy_spec.enthalpy  p_init_2P=0.101325 MPa  T_init_2P=293.15 K  x_init_2P=0.5  alpha_init_2P=0.5  h_init_2P=1500 kJ/kg  u_init_2P=1500 kJ/kg  mdot_nominal_TL=0.2 kg/s  delta_p_nominal_TL=0.01 MPa  p_in_nominal_TL=0.101325 MPa  T_in_nominal_TL=30 degC  volume_TL=0.001 m^3  nominal_init_TL=true  p_init_TL=0.101325 MPa  T_init_TL=293.15 K  a_liq_2P=0.023  a_mix_2P=0.005  a_vap_2P=0.023  b_2P=0.8  c_2P=0.33  a_TL=0.023  b_TL=0.8  c_TL=0.33
      settings: InternalSimscapePortConfiguration="{\"Bottom\":[],\"Left\":[{\"id\":\"A1\",\"label\":\"A1\",\"type\":\"foundation.two_phase_fluid.two_phase_fluid\"},{\"id\":\"B1\",\"label\":\"B1\",\"type\":\"foundation.two_phase_fluid.two_phase_fluid\"}],\"Right\":[{\"id\":\"A2\",\"label\":\"A2\",\"type\":\"foundation.thermal_liquid.thermal_liquid\"},{\"id\":\"B2\",\"label\":\"B2\",\"type\":\"foundation.thermal_liquid.thermal_liquid\"}],\"Top\":[{\"id\":\"Q1\",\"label\":\"Q1\",\"type\":\"output\"},{\"id\":\"Q2\",\"label\":\"Q2\",\"type\":\"output\"}]}"
  System-Level Heat Exchanger (TL-MA)1 : SimscapeFluids_lib/Heat Exchangers/Thermal Liquid - Moist Air/System-Level Heat Exchanger (TL-MA)  flow_arrangement=fluids.heat_exchangers.enum.SystemLevelFlowArrangementTLMA.Counter  wall_thermal_mass=false  mass_wall=1 kg  cp_wall=490 J/(K*kg)  nominal_init_wall=true  T_wall_init=293.15 K  area_A1=0.01 m^2  area_B1=0.01 m^2  area_A2=0.01 m^2  area_B2=0.01 m^2  operating_condition_TL=fluids.heat_exchangers.enum.SystemLevelOperatingConditionTLMA.Heating  mdot_nominal_TL=0.8 kg/s  delta_p_nominal_TL=0.01 MPa  p_in_nominal_TL=0.101325 MPa  T_in_nominal_TL=10 degC  capacity_spec_TL=fluids.heat_exchangers.enum.SystemLevelCapacitySpec.HeatTransfer  Q_nominal=2 kW  T_out_nominal_TL=323.15 K  volume_TL=0.001 m^3  nominal_init_TL=true  p_init_TL=0.101325 MPa  T_init_TL=293.15 K  mdot_nominal_MA=0.44 kg/s  delta_p_nominal_MA=0.001 MPa  p_in_nominal_MA=0.101325 MPa  T_in_nominal_MA=20.7 degC  inlet_humidity_spec_MA=foundation.enum.HumiditySpec.RelativeHumidity  RH_in_nominal_MA=0.5  x_w_in_nominal_MA=0.01  y_w_in_nominal_MA=0.01  HR_in_nominal_MA=0.01  Tw_in_nominal_MA=287 K  inlet_trace_gas_spec_MA=foundation.enum.trace_gas_spec.mass_fraction  x_g_in_nominal_MA=0.001  y_g_in_nominal_MA=0.001  volume_MA=0.1 m^3  nominal_init_MA=true  p_init_MA=0.101325 MPa  T_init_MA=293.15 K  humidity_spec_MA=foundation.enum.HumiditySpec.RelativeHumidity  RH_init_MA=0.5  x_w_init_MA=0.01  y_w_init_MA=0.01  HR_init_MA=0.01  Tw_init_MA=287 K  trace_gas_spec_MA=foundation.enum.trace_gas_spec.mass_fraction  x_g_init_MA=0.001  y_g_init_MA=0.001  r_d_init_MA=0  RH_ws_MA=1  time_constant_cond_MA=1e-3 s  time_constant_evap_MA=1e-3 s  fraction_entrained_MA=1  a_TL=0.023  b_TL=0.8  c_TL=0.33  a_MA=0.023  b_MA=0.8  c_MA=0.33
      settings: InternalSimscapePortConfiguration="{\"Bottom\":[],\"Left\":[{\"id\":\"A1\",\"label\":\"A1\",\"type\":\"foundation.thermal_liquid.thermal_liquid\"},{\"id\":\"B1\",\"label\":\"B1\",\"type\":\"foundation.thermal_liquid.thermal_liquid\"}],\"Right\":[{\"id\":\"A2\",\"label\":\"A2\",\"type\":\"foundation.moist_air.moist_air\"},{\"id\":\"B2\",\"label\":\"B2\",\"type\":\"foundation.moist_air.moist_air\"}],\"Top\":[{\"id\":\"Q1\",\"label\":\"Q1\",\"type\":\"output\"},{\"id\":\"Q2\",\"label\":\"Q2\",\"type\":\"output\"},{\"id\":\"W\",\"label\":\"W\",\"type\":\"output\"}]}"
  TOU meter : PythonCode  OutputCode=|
      | def TOU(unit,Time):
      |     if Time>=9 and Time <22 :
      |         return unit *5.79
      |     else : return unit*4
      | output = TOU(unit,Time)
  TOU meter1 : PythonCode  OutputCode=|
      | def TOU(unit,Time):
      |     if Time>=9 and Time <22 :
      |         return unit *5.79
      |     else : return unit*4
      | output = TOU(unit,Time)
  TOU meter2 : PythonCode  OutputCode=|
      | def TOU(unit,Time):
      |     if Time>=9 and Time <22 :
      |         return unit *5.79
      |     else : return unit*4
      | output = TOU(unit,Time)
  TOU meter3 : PythonCode  OutputCode=|
      | def TOU(unit,Time):
      |     if Time>=9 and Time <22 :
      |         return unit *5.79
      |     else : return unit*4
      | output = TOU(unit,Time)
  Tank (TL)1 : SimscapeFluids_lib/Thermal Liquid/Tanks & Accumulators/Tank (TL)  Commented=on  num_inlet=fluids.thermal_liquid.tanks_accumulators.enum.NumInlet.Three  pressure_spec=fluids.thermal_liquid.tanks_accumulators.enum.TankPressureSpec.Atmospheric  tank_pressure=0.101325 MPa  volume_spec=fluids.thermal_liquid.tanks_accumulators.enum.TankVolumeSpec.Constant  tank_area=0.25 m^2  level_TLU=[0, 3, 5] m  volume_TLU=[0, 4, 6] m^3  inlet_height_A=0.1 m  inlet_area_A=0.01 m^2  inlet_heights_AB=[.1, .9] m  inlet_areas_AB=[.00202, .00202] m^2  inlet_heights_ABC=[.9, .1, .9] m  inlet_areas_ABC=[0.03*0.03*pi, 0.03*0.03*pi,0.03*0.03*pi] m^2  inlet_heights_ABCD=0.1 * ones(1, 4) m  inlet_areas_ABCD=0.01 * ones(1, 4) m^2  inlet_heights_ABCDE=0.1 * ones(1, 5) m  inlet_areas_ABCDE=0.01 * ones(1, 5) m^2  inlet_heights_ABCDEF=0.1 * ones(1, 6) m  inlet_areas_ABCDEF=0.01 * ones(1, 6) m^2  level_check=simscape.enum.assert.action.error  capacity_check=simscape.enum.assert.action.none  max_capacity=10 m^3  g=9.81 m/s^2  level_specify=on  level_priority=None  level=1 m  level_nominal_specify=on  level_nominal_value=1  level_nominal_unit=m  volume_specify=off  volume_priority=None  volume=5 m^3  volume_nominal_specify=off  volume_nominal_value=1  volume_nominal_unit=m^3  mass_specify=on  mass_priority=Low  mass=250 kg  mass_nominal_specify=off  mass_nominal_value=1  mass_nominal_unit=kg  T_I_specify=on  T_I_priority=High  T_I=T_Tank_int_c degC  T_I_nominal_specify=off  T_I_nominal_value=1  T_I_nominal_unit=K
      settings: InternalSimscapePortConfiguration="{\"Bottom\":[{\"id\":\"H\",\"label\":\"H\",\"type\":\"foundation.thermal.thermal\"},{\"id\":\"T_out\",\"label\":\"T\",\"type\":\"output\"}],\"Left\":[{\"id\":\"A\",\"label\":\"A\",\"type\":\"foundation.thermal_liquid.thermal_liquid\"},{\"id\":\"B\",\"label\":\"B\",\"type\":\"foundation.thermal_liquid.thermal_liquid\"},{\"id\":\"C\",\"label\":\"C\",\"type\":\"foundation.thermal_liquid.thermal_liquid\"}],\"Right\":[],\"Top\":[{\"id\":\"V_out\",\"label\":\"V\",\"type\":\"output\"},{\"id\":\"L_out\",\"label\":\"L\",\"type\":\"output\"}]}"
  Tank (TL)2 : SimscapeFluids_lib/Thermal Liquid/Tanks & Accumulators/Tank (TL)  num_inlet=fluids.thermal_liquid.tanks_accumulators.enum.NumInlet.Three  pressure_spec=fluids.thermal_liquid.tanks_accumulators.enum.TankPressureSpec.Atmospheric  tank_pressure=0.101325 MPa  volume_spec=fluids.thermal_liquid.tanks_accumulators.enum.TankVolumeSpec.Constant  tank_area=0.25 m^2  level_TLU=[0, 3, 5] m  volume_TLU=[0, 4, 6] m^3  inlet_height_A=0.1 m  inlet_area_A=0.01 m^2  inlet_heights_AB=[.1, .9] m  inlet_areas_AB=[.00202, .00202] m^2  inlet_heights_ABC=[.9, .1, .9] m  inlet_areas_ABC=[0.03*0.03*pi, 0.03*0.03*pi,0.03*0.03*pi] m^2  inlet_heights_ABCD=0.1 * ones(1, 4) m  inlet_areas_ABCD=0.01 * ones(1, 4) m^2  inlet_heights_ABCDE=0.1 * ones(1, 5) m  inlet_areas_ABCDE=0.01 * ones(1, 5) m^2  inlet_heights_ABCDEF=0.1 * ones(1, 6) m  inlet_areas_ABCDEF=0.01 * ones(1, 6) m^2  level_check=simscape.enum.assert.action.error  capacity_check=simscape.enum.assert.action.none  max_capacity=10 m^3  g=9.81 m/s^2  level_specify=on  level_priority=None  level=1 m  level_nominal_specify=on  level_nominal_value=1  level_nominal_unit=m  volume_specify=off  volume_priority=None  volume=5 m^3  volume_nominal_specify=off  volume_nominal_value=1  volume_nominal_unit=m^3  mass_specify=on  mass_priority=Low  mass=250 kg  mass_nominal_specify=off  mass_nominal_value=1  mass_nominal_unit=kg  T_I_specify=on  T_I_priority=High  T_I=T_Tank_int_c-0 degC  T_I_nominal_specify=off  T_I_nominal_value=1  T_I_nominal_unit=K
      settings: InternalSimscapePortConfiguration="{\"Bottom\":[{\"id\":\"H\",\"label\":\"H\",\"type\":\"foundation.thermal.thermal\"},{\"id\":\"T_out\",\"label\":\"T\",\"type\":\"output\"}],\"Left\":[{\"id\":\"A\",\"label\":\"A\",\"type\":\"foundation.thermal_liquid.thermal_liquid\"},{\"id\":\"B\",\"label\":\"B\",\"type\":\"foundation.thermal_liquid.thermal_liquid\"},{\"id\":\"C\",\"label\":\"C\",\"type\":\"foundation.thermal_liquid.thermal_liquid\"}],\"Right\":[],\"Top\":[{\"id\":\"V_out\",\"label\":\"V\",\"type\":\"output\"},{\"id\":\"L_out\",\"label\":\"L\",\"type\":\"output\"}]}"
  Temperature Sensor : fl_lib/Thermal/Thermal Sensors/Temperature Sensor  temperature_measure=foundation.enum.MeasurementReference.difference
  Temperature Source : fl_lib/Thermal/Thermal Sources/Temperature Source  temperature=28 degC
  Thermal Liquid Properties (TL)1 : SimscapeFluids_lib/Thermal Liquid/Utilities/Thermal Liquid Properties (TL)  Commented=on  fluid_list=fluids.thermal_liquid.utilities.enum.thermal_liquid_fluid_list.water  concentration_param_EG=fluids.thermal_liquid.utilities.enum.thermal_liquid_concentration.volume_fraction  concentration_param_PG=fluids.thermal_liquid.utilities.enum.thermal_liquid_concentration.volume_fraction  c_mass_SW=3.5e-3  c_mass_EG=0.1  c_mass_PG=0.1  c_mass_GL=0.1  c_vol_EG=0.1  c_vol_PG=0.1  beta_const_EG=2.1791 GPa  beta_const_PG=2.1791 GPa  beta_const_GL=2.1791 GPa  p_min_EG=0.01 MPa  p_min_PG=0.01 MPa  p_min_GL=0.01 MPa  p_max_EG=50 MPa  p_max_PG=50 MPa  p_max_GL=50 MPa  p_atm=0.101325 MPa  properties_range_check=simscape.enum.assert.action.error
  Thermal Reference : fl_lib/Thermal/Thermal Elements/Thermal Reference
  Thermal Reference{1..6} (6 alike) : fl_lib/Thermal/Thermal Elements/Thermal Reference  Commented=on
  Thermostatic Expansion Valve (2P) : SimscapeFluids_lib/Two-Phase Fluid/Valves & Orifices/Flow Control Valves/Thermostatic Expansion Valve (2P)  valve_parameterization=fluids.two_phase_fluid.valves_orifices.flow_control_valves.enum.ThermostaticExpansionValveParameterization.Nominal  capacity_spec=fluids.two_phase_fluid.valves_orifices.flow_control_valves.enum.ThermostaticExpansionValveCapacitySpec.HeatTransfer  Q_nominal=m_dot*(h1-h4) kW  Q_max=m_dot*(h1-h4)+0.5 kW  mdot_nominal=0.005 kg/s  mdot_max=0.008 kg/s  pressure_spec=fluids.two_phase_fluid.valves_orifices.flow_control_valves.enum.ThermostaticExpansionValvePressureSpec.Pressure  p_cond_nominal=P3 MPa  p_evap_nominal=P1 MPa  T_cond_nominal=333.15 K  T_evap_nominal=273.15 K  delta_T_sub=1 deltaK  delta_T_nominal=5 deltaK  delta_T_static=4 deltaK  mop=fluids.two_phase_fluid.valves_orifices.flow_control_valves.enum.ThermostaticExpansionValveMOP.Off  p_mop=0.5 MPa  T_mop=288.15 K  T_evap_out_TLU1=0 : 10 : 40 degC  p_bulb_TLU1=0.3 : 0.1 : 0.7 MPa  lift_TLU2=0 : 0.15 : 0.6 mm  p_evap_TLU2=0.3 : -0.05 : 0.1 MPa  lift_TLU3=0 : 0.15 : 0.6 mm  mdot_TLU3=[1e-7, 0.015 : 0.015 : 0.06] kg/s  p_cond_ref=2 MPa  p_evap_ref=0.3 MPa  T_evap_out_ref=0 degC  delta_T_sub_ref=5 deltaK  pressure_equalization=fluids.two_phase_fluid.valves_orifices.flow_control_valves.enum.ThermostaticExpansionValveEqualization.Internal  bulb_dynamics=false  tau_bulb=20 s  leakage_fraction=1e-6  smoothing_factor=0.01  B_lam=0.999  tau_x=0.1 s  area=0.01 m^2
      settings: InternalSimscapePortConfiguration="{\"Bottom\":[],\"Left\":[{\"id\":\"A\",\"label\":\"A\",\"type\":\"foundation.two_phase_fluid.two_phase_fluid\"}],\"Right\":[{\"id\":\"B\",\"label\":\"B\",\"type\":\"foundation.two_phase_fluid.two_phase_fluid\"}],\"Top\":[{\"id\":\"S\",\"label\":\"S\",\"type\":\"foundation.two_phase_fluid.two_phase_fluid\"}]}"
  Thermostatic Expansion Valve (2P)1 : SimscapeFluids_lib/Two-Phase Fluid/Valves & Orifices/Flow Control Valves/Thermostatic Expansion Valve (2P)  valve_parameterization=fluids.two_phase_fluid.valves_orifices.flow_control_valves.enum.ThermostaticExpansionValveParameterization.Nominal  capacity_spec=fluids.two_phase_fluid.valves_orifices.flow_control_valves.enum.ThermostaticExpansionValveCapacitySpec.HeatTransfer  Q_nominal=3 kW  Q_max=4 kW  mdot_nominal=0.005 kg/s  mdot_max=0.008 kg/s  pressure_spec=fluids.two_phase_fluid.valves_orifices.flow_control_valves.enum.ThermostaticExpansionValvePressureSpec.Pressure  p_cond_nominal=P3 MPa  p_evap_nominal=P1 MPa  T_cond_nominal=333.15 K  T_evap_nominal=273.15 K  delta_T_sub=1 deltaK  delta_T_nominal=6 deltaK  delta_T_static=5 deltaK  mop=fluids.two_phase_fluid.valves_orifices.flow_control_valves.enum.ThermostaticExpansionValveMOP.Off  p_mop=0.5 MPa  T_mop=288.15 K  T_evap_out_TLU1=0 : 10 : 40 degC  p_bulb_TLU1=0.3 : 0.1 : 0.7 MPa  lift_TLU2=0 : 0.15 : 0.6 mm  p_evap_TLU2=0.3 : -0.05 : 0.1 MPa  lift_TLU3=0 : 0.15 : 0.6 mm  mdot_TLU3=[1e-7, 0.015 : 0.015 : 0.06] kg/s  p_cond_ref=2 MPa  p_evap_ref=0.3 MPa  T_evap_out_ref=0 degC  delta_T_sub_ref=5 deltaK  pressure_equalization=fluids.two_phase_fluid.valves_orifices.flow_control_valves.enum.ThermostaticExpansionValveEqualization.Internal  bulb_dynamics=false  tau_bulb=20 s  leakage_fraction=1e-6  smoothing_factor=0.01  B_lam=0.999  tau_x=0.1 s  area=0.01 m^2
      settings: InternalSimscapePortConfiguration="{\"Bottom\":[],\"Left\":[{\"id\":\"A\",\"label\":\"A\",\"type\":\"foundation.two_phase_fluid.two_phase_fluid\"}],\"Right\":[{\"id\":\"B\",\"label\":\"B\",\"type\":\"foundation.two_phase_fluid.two_phase_fluid\"}],\"Top\":[{\"id\":\"S\",\"label\":\"S\",\"type\":\"foundation.two_phase_fluid.two_phase_fluid\"}]}"
  To Workspace : ToWorkspace  VariableName=V_Discharge  SaveFormat=Timeseries  SampleTime=1
  To Workspace1 : ToWorkspace  VariableName=V_Main  SaveFormat=Timeseries  SampleTime=1
  To Workspace10 : ToWorkspace  VariableName=Q_Evap  SaveFormat=Timeseries  SampleTime=1
  To Workspace11 : ToWorkspace  VariableName=Q_House  SaveFormat=Timeseries  SampleTime=1
  To Workspace12 : ToWorkspace  VariableName=Q_Room  SaveFormat=Timeseries  SampleTime=1
  To Workspace13 : ToWorkspace  VariableName=Q_Charge  SaveFormat=Timeseries  SampleTime=1
  To Workspace14 : ToWorkspace  VariableName=Q_Load  SaveFormat=Timeseries  SampleTime=1
  To Workspace15 : ToWorkspace  VariableName=P_FanEvap  SaveFormat=Timeseries  SampleTime=1
  To Workspace16 : ToWorkspace  VariableName=P_Compsr  SaveFormat=Timeseries  SampleTime=1
  To Workspace17 : ToWorkspace  VariableName=P_FanCond  SaveFormat=Timeseries  SampleTime=1
  To Workspace18 : ToWorkspace  VariableName=P_Pump  SaveFormat=Timeseries  SampleTime=1
  To Workspace19 : ToWorkspace  VariableName=N_People  SaveFormat=Timeseries  SampleTime=1
  To Workspace2 : ToWorkspace  VariableName=V_R32  SaveFormat=Timeseries  SampleTime=1
  To Workspace20 : ToWorkspace  VariableName=Cost_FanEvap  SaveFormat=Timeseries  SampleTime=1
  To Workspace21 : ToWorkspace  VariableName=Cost_FanCond  SaveFormat=Timeseries  SampleTime=1
  To Workspace22 : ToWorkspace  VariableName=Cost_Compsr  SaveFormat=Timeseries  SampleTime=1
  To Workspace23 : ToWorkspace  VariableName=Cost_Pump  SaveFormat=Timeseries  SampleTime=1
  To Workspace24 : ToWorkspace  VariableName=Cost_Total  SaveFormat=Timeseries  SampleTime=1
  To Workspace3 : ToWorkspace  VariableName=Stat_Compsr  SaveFormat=Timeseries  SampleTime=1
  To Workspace4 : ToWorkspace  VariableName=Stat_FanEvap  SaveFormat=Timeseries  SampleTime=1
  To Workspace5 : ToWorkspace  VariableName=Stat_FanCond  SaveFormat=Timeseries  SampleTime=1
  To Workspace6 : ToWorkspace  VariableName=Stat_Pump  SaveFormat=Timeseries  SampleTime=1
  To Workspace7 : ToWorkspace  VariableName=T_Room  SaveFormat=Timeseries  SampleTime=1
  To Workspace8 : ToWorkspace  VariableName=T_WaterTank  SaveFormat=Timeseries  SampleTime=1
  To Workspace9 : ToWorkspace  VariableName=Q_Cond  SaveFormat=Timeseries  SampleTime=1
  Transfer Fcn2 : TransferFcn  Denominator=[1 1]
  Transfer Fcn{3..6} (4 alike) : TransferFcn  Denominator=[4 1]
  Transfer Fcn7 : TransferFcn  Denominator=[1 1]
  Transfer Fcn8 : TransferFcn  Denominator=[1 1]
  Wt : SimscapeFluids_lib/Thermal Liquid/Utilities/Thermal Liquid Properties (TL)  fluid_list=fluids.thermal_liquid.utilities.enum.thermal_liquid_fluid_list.water  concentration_param_EG=fluids.thermal_liquid.utilities.enum.thermal_liquid_concentration.volume_fraction  concentration_param_PG=fluids.thermal_liquid.utilities.enum.thermal_liquid_concentration.volume_fraction  c_mass_SW=3.5e-3  c_mass_EG=0.1  c_mass_PG=0.1  c_mass_GL=0.1  c_vol_EG=0.1  c_vol_PG=0.1  beta_const_EG=2.1791 GPa  beta_const_PG=2.1791 GPa  beta_const_GL=2.1791 GPa  p_min_EG=0.01 MPa  p_min_PG=0.01 MPa  p_min_GL=0.01 MPa  p_max_EG=50 MPa  p_max_PG=50 MPa  p_max_GL=50 MPa  p_atm=0.101325 MPa  properties_range_check=simscape.enum.assert.action.error
  tag scope: Cost_Compsr=global, Cost_FanCond=global, Cost_FanEvap=global, Cost_Pump=global, Cost_Total=global, Hr=global, P_Compsr_kW=global, P_FanCond_kW=global, P_FanEvap_kW=global, Q_Cond=global, Q_Discharge=global, Q_Evap=global, Q_House=global, Room_Temp=global, STAT=global, T_MA_Evap=global, T_MA_wtCoil=global, T_Tank=global, Unit_Compsr=global, Unit_FanCond=global, Unit_FanEvap=global, Unit_Pump=global, V_Discharge=global, V_main=global, V_r32=global, f_MA_return=global, f_water_Charge=global, f_water_Discharge=global, f_water_main=global, n_Light=global, n_laptop=global, n_people=global, n_projector=global, on_off_Conpsr=global, on_off_FanCond=global, on_off_FanEvap=global, on_off_Pump=global
  wires:
  PS-Simulink Converter1/1 -> [Q_Evap]
  PS-Simulink Converter/1 -> [Q_Cond]
  PS-Simulink Converter6/1 -> [Q_House]
  PS-Simulink Converter4/1 -> [Room_Temp]
  Transfer Fcn6/1 -> [on_off_Conpsr]
  Transfer Fcn3/1 -> [on_off_FanEvap]
  Transfer Fcn4/1 -> [on_off_FanCond]
  [f_r32_Evap] -> Mux/3  "fr-r32-Evap"
  [f_r32_TES] -> Mux/2  "fr-r32-TES"
  [f_r32_main] -> Mux/1  "fr-r32-main"
  PS-Simulink Converter5/1 -> [f_MA_return]
  Transfer Fcn2/1 -> [V_r32]
  [Q_Cond] -> Mux2/1  "Q_Cond : kW"
  [Q_Evap] -> Mux2/2  "Q_Evap : kW"
  [Q_Discharge] -> Mux2/3  "Q_Discharge : kW"
  [Q_House] -> Mux2/4  "Q_House : kW"
  [Q_Load] -> Mux2/5  "Q_Load : kW"
  PS-Simulink Converter8/1 -> [Q_Load]
  Transfer Fcn5/1 -> [on_off_Pump]
  PS-Simulink Converter2/1 -> Goto14/1
  PS-Simulink Converter3/1 -> [Q_Discharge]
  [f_MA_Evap] -> Mux3/1  "f_MA_Evap"
  Q_Charge/1(Q) -> Mux2/6  "Q_Charge : kW"
  From6/1 -> Simulink-PS Converter/1
  [f_MA_WaterCoil] -> Mux3/2  "f_MA_wtCoil"
  [f_water_main] -> Mux4/1  "f_water_main"
  [f_water_Charge] -> Mux4/2  "f_water_Charge"
  [f_water_Discharge] -> Mux4/3  "f_water_Discharge"
  Mux/1 -> Scope/1
  Mux2/1 -> Scope/2
  Mux3/1 -> Scope/3
  Mux4/1 -> Scope/4
  [Room_Temp] -> Mux5/2  "Room : degC"
  [T_Tank] -> Mux5/1  "Tank : degC"
  Mux5/1 -> Scope/5
  From24/1 -> Relay/1
  Relay/1 -> Simulink-PS Converter2/1
  [T_in] -> Mux6/1  "T_r32_in : degC"
  [T_out] -> Mux6/2  "T_r32_out :degC"
  Mux6/1 -> Scope/6
  [V_main] -> Simulink-PS Converter3/1
  [V_Discharge] -> Simulink-PS Converter7/1
  PS-Simulink Converter7/1 -> [f_water_main]
  PS-Simulink Converter9/1 -> [f_water_Charge]
  PS-Simulink Converter10/1 -> [f_water_Discharge]
  [on_off_Pump] -> Simulink-PS Converter9/1
  PS-Simulink Converter12/1 -> [T_Tank]
  [V_Discharge] -> Mux7/1  "V_Discharge"
  [V_main] -> Mux7/2  "V_main"
  Mux7/1 -> Scope/8
  Transfer Fcn7/1 -> [V_Discharge]
  Transfer Fcn8/1 -> [V_main]
  [on_off_Conpsr] -> Mux8/1  "Compsr_Stat"
  [on_off_FanEvap] -> Mux8/2  "FanEvap_Stat"
  Mux8/1 -> Scope/9
  [T_Tank] -> Chart1/2(T_tank)  "T_r32_in : degC"
  [T_Tank] -> Chart1/1(T_Tank)  "Tank : degC"
  From22/1 -> Gain6/1
  From19/1 -> Gain3/1
  From13/1 -> Gain1/1
  Gain1/1 -> Simulink-PS Converter4/1  "*10watt/unit"
  Gain6/1 -> Gain5/1  "Number"
  Gain4/1 -> Simulink-PS Converter5/1  "*10watt/unit"
  Gain5/1 -> Simulink-PS Converter6/1  "*10watt/unit"
  Gain3/1 -> Simulink-PS Converter1/1  "*10watt/unit"
  From21/1 -> Gain7/1
  Gain7/1 -> Gain4/1  "Number"
  Gain2/1 -> Simulink-PS Converter8/1  "*10watt/unit"
  Constant3/1 -> Gain20/1
  Constant2/1 -> Gain2/1
  Gain20/1 -> Simulink-PS Converter10/1  "*10watt/unit"
  [on_off_FanCond] -> Integrator4/1
  [P_Compsr_kW] -> Display7/1  "kW"
  [Unit_FanCond] -> Display9/1  "kWh"
  [Unit_Compsr] -> TOU meter2/1
  [on_off_FanEvap] -> Integrator3/1
  Gain10/1 -> [Unit_FanCond]
  [Hr] -> TOU meter1/2
  [Hr] -> TOU meter2/2
  [P_FanCond_kW] -> Integrator1/1  "kW"
  [on_off_Conpsr] -> Gain9/1
  [P_Compsr_kW] -> Integrator2/1  "kW"
  [on_off_FanEvap] -> Gain8/1
  Gain12/1 -> [Unit_FanEvap]
  [on_off_FanCond] -> Gain/1
  Gain9/1 -> [P_Compsr_kW]  "kW"
  [P_FanEvap_kW] -> Display5/1  "kW"
  Integrator1/1 -> Gain10/1  "kWs"
  TOU meter1/1 -> [Cost_FanCond], Add/3  "Costs"
  [Hr] -> TOU meter/2
  Gain11/1 -> [Unit_Compsr]
  Integrator2/1 -> Gain11/1  "kWs"
  [on_off_Conpsr] -> Integrator5/1
  Integrator4/1 -> Display3/1  "sec"
  Gain/1 -> [P_FanCond_kW]  "kW"
  TOU meter/1 -> [Cost_FanEvap], Add/4  "Costs"
  [Unit_FanCond] -> TOU meter1/1
  [Unit_FanEvap] -> TOU meter/1
  Integrator/1 -> Gain12/1  "kWs"
  Integrator5/1 -> Display4/1  "sec"
  [P_FanEvap_kW] -> Integrator/1  "kW"
  [Unit_Compsr] -> Display10/1  "kWh"
  [Unit_FanEvap] -> Display8/1  "kWh"
  Integrator3/1 -> Display/1  "sec"
  [P_FanCond_kW] -> Display6/1  "kW"
  Add/1 -> [Cost_Total]
  Gain8/1 -> [P_FanEvap_kW]  "kW"
  Saturation/1 -> [n_laptop], [n_Light]
  From Spreadsheet/6 -> [n_projector], [n_people], Saturation/1
  From Spreadsheet/1 -> [Hr]
  23-12-2025/1(Out1) -> [STAT]  "Switch"
  Chart2/2(Cond) -> Transfer Fcn4/1
  Chart2/3(Evap) -> Transfer Fcn3/1
  Chart2/4(Pump) -> Transfer Fcn5/1
  Chart2/5(V_R32) -> Transfer Fcn2/1
  Chart2/7(V_main) -> Transfer Fcn8/1
  Chart2/6(V_discharge) -> Transfer Fcn7/1
  [T_Tank] -> Chart2/1(T_Tank)  "Tank"
  [Room_Temp] -> Chart2/2(T_Room)  "Room"
  Chart2/1(Comp) -> Transfer Fcn6/1
  [V_r32] -> Mux7/3  "V_R32"
  [on_off_Pump] -> Mux8/3  "Pump_Stat"
  Mux1/1 -> Scope/7
  PS-Simulink Converter11/1 -> [T_MA_Evap]
  PS-Simulink Converter13/1 -> [T_MA_wtCoil]
  [T_MA_Evap] -> Mux1/1  "T_MA_EVAP"
  [T_MA_wtCoil] -> Mux1/2  "T_MA_wtCoil"
  [Q_House] -> To Workspace11/1  "Q_House : kW"
  Q_Charge1/1(Q) -> To Workspace13/1  "Q_Charge : kW"
  [Q_Load] -> To Workspace14/1  "Q_Load : kW"
  [Q_Discharge] -> To Workspace12/1  "Q_Discharge : kW"
  [Q_Evap] -> To Workspace10/1  "Q_Evap : kW"
  [Q_Cond] -> To Workspace9/1  "Q_Cond : kW"
  [V_Discharge] -> To Workspace/1
  [V_main] -> To Workspace1/1
  [V_r32] -> To Workspace2/1
  [on_off_Conpsr] -> To Workspace3/1
  [on_off_FanEvap] -> To Workspace4/1
  [on_off_FanCond] -> To Workspace5/1
  [on_off_Pump] -> To Workspace6/1
  [Room_Temp] -> To Workspace7/1
  [T_Tank] -> To Workspace8/1
  [P_FanEvap_kW] -> To Workspace15/1  "kW"
  [P_FanCond_kW] -> To Workspace17/1  "kW"
  [P_Compsr_kW] -> To Workspace16/1  "kW"
  [P_Pump_kW] -> To Workspace18/1  "kW"
  [on_off_Pump] -> Gain13/1
  Gain13/1 -> [P_Pump_kW]  "kW"
  [n_people] -> To Workspace19/1
  [Hr] -> TOU meter3/2
  [Unit_Pump] -> TOU meter3/1
  TOU meter2/1 -> [Cost_Compsr], Add/2  "Costs"
  TOU meter3/1 -> [Cost_Pump], Add/1  "Costs"
  [Cost_FanCond] -> Display12/1
  [Cost_FanEvap] -> Display11/1
  [Cost_Pump] -> Display14/1
  [Cost_Compsr] -> Display13/1
  Gain14/1 -> [Unit_Pump]
  [P_Pump_kW] -> Integrator6/1  "kW"
  Integrator6/1 -> Gain14/1  "kWs"
  [Unit_Pump] -> Display1/1  "kWh"
  [on_off_Pump] -> Integrator7/1
  Integrator7/1 -> Display2/1  "sec"
  [P_Pump_kW] -> Display15/1  "kW"
  [Cost_Total] -> Display16/1
  [Cost_Compsr] -> To Workspace22/1
  [Cost_FanEvap] -> To Workspace20/1
  [Cost_FanCond] -> To Workspace21/1
  [Cost_Pump] -> To Workspace23/1
  [Cost_Total] -> To Workspace24/1
  connections:
  Constant Volume Chamber (MA)/LConn2 -- Fan (MA)/LConn1
  Solver Configuration/RConn1 -- R32/RConn1 -- Flow Resistance (2P)/RConn1 -- S3/LConn1 -- Condenser/LConn2
  Evaporator/LConn2 -- Thermostatic Expansion Valve (2P)/LConn2 -- S1/LConn1 -- Subsystem/LConn1
  Evaporator/LConn1 -- Thermostatic Expansion Valve (2P)/RConn1 -- S5/LConn1
  Evaporator/RConn2 -- Pressure & Temperature Sensor (MA)/LConn1 -- Flow Rate Sensor (MA)1/LConn1
  Receiver Accumulator (2P)/RConn2 -- Flow Resistance (2P)/LConn1
  Condenser/LConn4 -- PS-Simulink Converter/LConn1
  Evaporator/LConn3 -- PS-Simulink Converter1/LConn1
  Temperature Sensor/RConn1 -- Thermal Reference/LConn1
  Amplifier/LConn1 -- Laptop Charge/LConn1 -- Laptop/LConn1 -- Occupants/LConn1 -- Heat Flow Rate Sensor1/LConn1 -- Projector/LConn1 -- Lights/LConn1
  PS-Simulink Converter4/LConn1 -- Temperature Sensor/RConn2
  PS-Simulink Converter5/LConn1 -- Flow Rate Sensor (MA)1/RConn2
  Flow Rate Sensor (MA)1/RConn1 -- Constant Volume Chamber (MA)/LConn3
  PS-Simulink Converter6/LConn1 -- Heat Flow Rate Sensor/RConn1
  House Thermal Network/RConn1 -- Heat Flow Rate Sensor/LConn1
  House Thermal Network/LConn1 -- Temperature Source/LConn1
  Enviroment/LConn1 -- Condenser/RConn2
  Condenser/RConn1 -- Enviroment/RConn1
  Heat Flow Rate Sensor/RConn2 -- Heat Flow Rate Sensor1/RConn2 -- Temperature Sensor/LConn1 -- Constant Volume Chamber (MA)/RConn3
  PS-Simulink Converter8/LConn1 -- Heat Flow Rate Sensor1/RConn1
  S4/LConn1 -- Control Valve R32/RConn2 -- Thermostatic Expansion Valve (2P)/LConn1
  Control Valve R32/LConn1 -- Receiver Accumulator (2P)/LConn2
  Condenser/LConn1 -- "Flow rate sensor : R32"/RConn1 -- S2/LConn1
  Positive-Displacement Compressor (2P)/RConn1 -- "Flow rate sensor : R32"/LConn1
  Subsystem/LConn2 -- Positive-Displacement Compressor (2P)/LConn1
  PS-Simulink Converter2/LConn1 -- Tank (TL)1/RConn2
  Pipe (TL)3/LConn1 -- Tank (TL)1/LConn2
  Centrifugal Pump (TL)2/RConn2 -- Ideal Angular Velocity Source3/RConn2
  Centrifugal Pump (TL)2/LConn1 -- Pipe (TL)3/RConn1
  Pipe (TL)4/RConn1 -- Tank (TL)1/LConn3
  PS-Simulink Converter3/LConn1 -- System-Level Heat Exchanger (TL-MA)1/LConn3
  Moist Air Properties (MA)2/RConn1 -- Constant Volume Chamber (MA)/LConn1 -- Pressure & Temperature Sensor (MA)1/LConn1 -- System-Level Heat Exchanger (TL-MA)1/RConn2
  Tank (TL)1/LConn1 -- Pipe (TL)5/RConn1
  System-Level Condenser Evaporator (2P-TL)/RConn2 -- Check Valve (TL)/LConn1
  Inlet/RConn1 -- System-Level Condenser Evaporator (2P-TL)/LConn1 -- Thermostatic Expansion Valve (2P)1/RConn1
  Thermostatic Expansion Valve (2P)1/LConn1 -- Control Valve R32/RConn1
  Subsystem/RConn1 -- System-Level Condenser Evaporator (2P-TL)/LConn2 -- Thermostatic Expansion Valve (2P)1/LConn2 -- Outlet/LConn1
  Fan Drive/RConn1 -- Fan (MA)/LConn2
  Fan Drive/LConn1 -- Fan (MA)/RConn2
  Subsystem1/RConn2 -- Evaporator/RConn1
  Subsystem1/RConn1 -- System-Level Heat Exchanger (TL-MA)1/RConn1
  Fan (MA)/RConn1 -- Subsystem1/LConn1
  System-Level Condenser Evaporator (2P-TL)/RConn1 -- Flow Rate Sensor (TL)1/RConn1
  Centrifugal Pump (TL)2/LConn2 -- Subsystem2/LConn1
  PS Gain1/RConn1 -- Ideal Angular Velocity Source3/RConn1
  Simulink-PS Converter/RConn1 -- PS Gain1/LConn1
  Positive-Displacement Compressor (2P)/RConn2 -- Subsystem3/LConn1
  Subsystem3/RConn1 -- Positive-Displacement Compressor (2P)/LConn2
  Centrifugal Pump (TL)/LConn2 -- Flow Rate Sensor (TL)/LConn1
  Flow Rate Sensor (TL)1/LConn1 -- Master Valve/RConn3
  Master Valve/RConn2 -- Discharge Valve/LConn2
  Master Valve/LConn1 -- Flow Rate Sensor (TL)/RConn1
  Tank (TL)2/LConn2 -- Centrifugal Pump (TL)/LConn1
  Pipe (TL)1/RConn1 -- Wt/RConn1 -- Tank (TL)2/LConn1
  Tank (TL)2/LConn3 -- Pipe (TL)2/RConn1
  Master Valve/RConn1 -- Simulink-PS Converter3/RConn1
  Discharge Valve/RConn1 -- Pipe (TL)2/LConn1
  Check Valve (TL)1/RConn1 -- Discharge Valve/LConn3
  Simulink-PS Converter7/RConn1 -- Discharge Valve/LConn1
  System-Level Heat Exchanger (TL-MA)1/LConn2 -- Check Valve (TL)1/LConn1
  Flow Rate Sensor (TL)1/RConn2 -- PS-Simulink Converter9/LConn1
  Flow Rate Sensor (TL)2/RConn2 -- PS-Simulink Converter10/LConn1
  Flow Rate Sensor (TL)/RConn2 -- PS-Simulink Converter7/LConn1
  Flow Rate Sensor (TL)2/LConn1 -- Discharge Valve/RConn2
  Mechanical Rotational Reference1/LConn1 -- Centrifugal Pump (TL)/RConn1 -- Ideal Angular Velocity Source1/LConn1
  Simulink-PS Converter9/RConn1 -- PS Gain2/LConn1
  PS Gain2/RConn1 -- Ideal Angular Velocity Source1/RConn1
  Ideal Angular Velocity Source1/RConn2 -- Centrifugal Pump (TL)/RConn2
  PS-Simulink Converter12/LConn1 -- Tank (TL)2/RConn2
  System-Level Heat Exchanger (TL-MA)1/LConn1 -- Flow Rate Sensor (TL)2/RConn1
  Check Valve (TL)/RConn1 -- Pipe (TL)1/LConn1
  Simulink-PS Converter1/RConn1 -- Occupants/RConn1
  Lights/RConn2 -- Thermal Reference3/LConn1
  Occupants/RConn2 -- Thermal Reference1/LConn1
  Simulink-PS Converter4/RConn1 -- Projector/RConn1
  Simulink-PS Converter5/RConn1 -- Laptop/RConn1
  Laptop/RConn2 -- Thermal Reference2/LConn1
  Projector/RConn2 -- Thermal Reference4/LConn1
  Simulink-PS Converter6/RConn1 -- Lights/RConn1
  Thermal Reference6/LConn1 -- Amplifier/RConn2
  Simulink-PS Converter8/RConn1 -- Laptop Charge/RConn1
  Thermal Reference5/LConn1 -- Laptop Charge/RConn2
  Simulink-PS Converter10/RConn1 -- Amplifier/RConn1
  Pressure & Temperature Sensor (MA)/RConn1 -- PS-Simulink Converter11/LConn1
  Pressure & Temperature Sensor (MA)1/RConn1 -- PS-Simulink Converter13/LConn1
